simulink model "MIL4L3_SW6_V1_20220211"  (R2018b)
settings: Solver=FixedStepAuto  StartTime=0.0  StopTime=inf  FixedStep=0.001  RelTol=1e-3
PreLoadFcn:
  | A0_MILtest;
undefined symbols (not defined in the file or in its folder): Clb_ICADirect_LaneDisp_StateFive, Clb_ICADirect_LaneDisp_StateFour, Clb_ICADirect_LaneDisp_StateOne, Clb_ICADirect_LaneDisp_StateThree, Clb_ICADirect_LaneDisp_StateTwo, Clb_ICADirect_LaneDisp_StateZero, Clb_ICADirect_LaneDispSW, Clb_ICADirect_TrnLghtsCom_Switch, Clb_ICADirect_TrnLghtsCom_Value, Clb_ICADirect_TrnLghtsCrtl_Inhb, IMAP_Clb_ACU_Driver_Belt, IMAP_Clb_ACU_Driver_Belt_Over, IMAP_Clb_ACU_Passenger_Belt, IMAP_Clb_ACU_Passenger_Belt_Over, IMAP_Clb_ACU_RearLeft_Belt, IMAP_Clb_ACU_RearLeft_Belt_Over, IMAP_Clb_ACU_RearMiddle_Belt, IMAP_Clb_ACU_RearMiddle_Belt_Over, IMAP_Clb_ACU_RearRight_Belt, IMAP_Clb_ACU_RearRight_Belt_Over, IMAP_Clb_AEB_Switch, IMAP_Clb_AEB_Switch_Over, IMAP_Clb_ALC_TLC_Mode, IMAP_Clb_ALC_TLC_Mode_Over, IMAP_Clb_BCM_Battery_Voltage, IMAP_Clb_BCM_Battery_Voltage_Over, IMAP_Clb_BCM_BrakeLamp_State, IMAP_Clb_BCM_BrakeLamp_State_Over, IMAP_Clb_BCM_CHMSL_Status, IMAP_Clb_BCM_CHMSL_Status_Over, IMAP_Clb_BCM_Door_Lock_State, IMAP_Clb_BCM_Door_Lock_State_Over, IMAP_Clb_BCM_FrontWiper_State, IMAP_Clb_BCM_FrontWiper_State_Over, IMAP_Clb_BCM_FrontWiper_Switch, IMAP_Clb_BCM_FrontWiper_Switch_Over, IMAP_Clb_BCM_HazardLamp, IMAP_Clb_BCM_HazardLamp_Over, IMAP_Clb_BCM_HazardLamp_Switch, IMAP_Clb_BCM_HazardLamp_Switch_Over, IMAP_Clb_BCM_HighBeam_State, IMAP_Clb_BCM_HighBeam_State_Over, IMAP_Clb_BCM_Ignition_State, IMAP_Clb_BCM_Ignition_State_Over, IMAP_Clb_BCM_IHBC_Enabled, IMAP_Clb_BCM_IHBC_Enabled_Over, IMAP_Clb_BCM_Left_Light, IMAP_Clb_BCM_Left_Light_Over, IMAP_Clb_BCM_LeftTurn_Switch, IMAP_Clb_BCM_LeftTurn_Switch_Over, IMAP_Clb_BCM_LF_Door_State, IMAP_Clb_BCM_LF_Door_State_Over, IMAP_Clb_BCM_LowBeam_State, IMAP_Clb_BCM_LowBeam_State_Over, IMAP_Clb_BCM_LR_Door_State, IMAP_Clb_BCM_LR_Door_State_Over, IMAP_Clb_BCM_RF_Door_State, IMAP_Clb_BCM_RF_Door_State_Over, IMAP_Clb_BCM_Right_Light, IMAP_Clb_BCM_Right_Light_Over ... (+547)
libraries: CarMaker4SL x2153, simulink x292, dspstat3 x3, canmsglib x2, simulink_extras x1
(part 28 of 52)

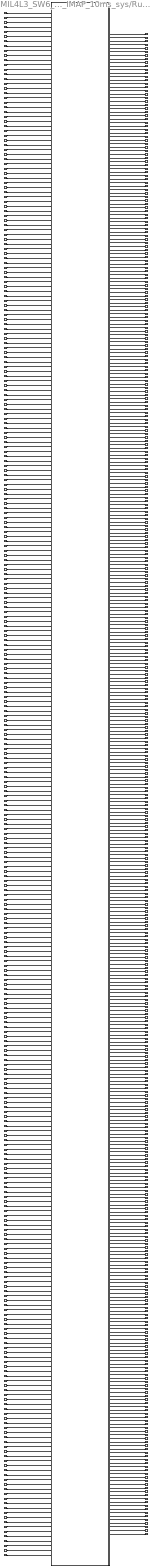
== system MIL4L3_SW6_V1_20220211/CarMaker/VehicleControl/Data Inport/IMAP/Runnable_IMAP_10ms_sys/Runnable_IMAP_10ms_sys ==
  SWINve_y_ABS_in_regulation : Inport  OutDataTypeStr=uint8  PortDimensions=1
  SWINve_g_ACCEL_LONGI_CALIB : Inport  Port=2  OutDataTypeStr=single  PortDimensions=1
  SWINve_y_ASR_ESP_disconnected : Inport  Port=3  OutDataTypeStr=uint8  PortDimensions=1
  SWINve_y_ASR_in_regulation : Inport  Port=4  OutDataTypeStr=uint8  PortDimensions=1
  SWINve_y_BCM_BrakeLampStatus : Inport  Port=5  OutDataTypeStr=uint8  PortDimensions=1
  SWINve_y_BCM_CHMSLStatus : Inport  Port=6  OutDataTypeStr=uint8  PortDimensions=1
  SWINve_y_BCM_State_Front_Wiper : Inport  Port=7  OutDataTypeStr=uint8  PortDimensions=1
  SWINve_y_BCM_Status_Indicator : Inport  Port=8  OutDataTypeStr=uint8  PortDimensions=1
  SWINve_y_Brake_secondary_contact : Inport  Port=9  OutDataTypeStr=uint8  PortDimensions=1
  SWINve_y_Braking_effort : Inport  Port=10  OutDataTypeStr=uint8  PortDimensions=1
  SWINve_y_Dynamic_slope : Inport  Port=11  OutDataTypeStr=int8  PortDimensions=1
  SWINve_y_Dynamic_slope_accuracy : Inport  Port=12  OutDataTypeStr=uint8  PortDimensions=1
  SWINve_y_EMS_ACC_Effecitive_EMS : Inport  Port=13  OutDataTypeStr=uint8  PortDimensions=1
  SWINve_y_EMS_ACCcontrol_Available : Inport  Port=14  OutDataTypeStr=uint8  PortDimensions=1
  SWINve_g_EMS_Acceleration_pedal_position : Inport  Port=15  OutDataTypeStr=single  PortDimensions=1
  SWINve_g_EMS_Actual_torque : Inport  Port=16  OutDataTypeStr=single  PortDimensions=1
  SWINve_g_EMS_Actual_whlTrq : Inport  Port=17  OutDataTypeStr=int16  PortDimensions=1
  SWINve_g_EMS_Driver_request : Inport  Port=18  OutDataTypeStr=single  PortDimensions=1
  SWINve_g_EMS_Driver_wheel_torque : Inport  Port=19  OutDataTypeStr=single  PortDimensions=1
  SWINve_g_EMS_Engine_RPM : Inport  Port=20  OutDataTypeStr=single  PortDimensions=1
  SWINve_y_EMS_Engine_state : Inport  Port=21  OutDataTypeStr=uint8  PortDimensions=1
  SWINve_y_EMS_GearBox_ACC_Ctl_Available : Inport  Port=22  OutDataTypeStr=uint8  PortDimensions=1
  SWINve_g_EMS_WhlTrq_max : Inport  Port=23  OutDataTypeStr=single  PortDimensions=1
  SWINve_g_EMS_WhlTrq_max_offset : Inport  Port=24  OutDataTypeStr=single  PortDimensions=1
  SWINve_g_EMS_WhlTrq_min : Inport  Port=25  OutDataTypeStr=single  PortDimensions=1
  SWINve_g_EMS_WhlTrq_min_offset : Inport  Port=26  OutDataTypeStr=single  PortDimensions=1
  SWINve_y_ESP_in_regulation : Inport  Port=27  OutDataTypeStr=uint8  PortDimensions=1
  SWINve_y_Front_Left_pulse_malfunction : Inport  Port=28  OutDataTypeStr=uint8  PortDimensions=1
  SWINve_y_Front_right_pulse_malfunction : Inport  Port=29  OutDataTypeStr=uint8  PortDimensions=1
  SWINve_y_GW_BCM_SEV_main_state : Inport  Port=30  OutDataTypeStr=uint8  PortDimensions=1
  SWINve_y_GW_EMS_ACC_Ihibited_By_Engine : Inport  Port=31  OutDataTypeStr=uint8  PortDimensions=1
  SWINve_y_GW_EMS_EMS_Status_ACC : Inport  Port=32  OutDataTypeStr=uint8  PortDimensions=1
  SWINve_g_GW_EMS_Pot_WhlTrq_Max : Inport  Port=33  OutDataTypeStr=single  PortDimensions=1
  SWINve_g_GW_EMS_Pot_WhlTrq_Min : Inport  Port=34  OutDataTypeStr=single  PortDimensions=1
  SWINve_y_GW_Mp5_ISA_Switch : Inport  Port=35  OutDataTypeStr=uint8  PortDimensions=1
  SWINve_y_GW_Mp5_TSR_Switch : Inport  Port=36  OutDataTypeStr=uint8  PortDimensions=1
  SWINve_y_GW_SCC_LeftSteeringWheelSwitch : Inport  Port=37  OutDataTypeStr=uint8  PortDimensions=1
  SWINve_y_GW_SCC_RightSteeringWheelSwitch : Inport  Port=38  OutDataTypeStr=uint8  PortDimensions=1
  SWINve_y_BCM_HazardSwitchrSt : Inport  Port=39  OutDataTypeStr=uint8  PortDimensions=1
  SWINve_y_MP5_HazardLampCtrlReq : Inport  Port=40  OutDataTypeStr=uint8  PortDimensions=1
  SWINve_y_T_box_RemoteHazardReq : Inport  Port=41  OutDataTypeStr=uint8  PortDimensions=1
  SWINve_y_High_beam_state : Inport  Port=42  OutDataTypeStr=uint8  PortDimensions=1
  SWINve_y_IC_Fcw_Activation_Config : Inport  Port=43  OutDataTypeStr=uint8  PortDimensions=1
  SWINve_y_IC_FCW_Sensitivity : Inport  Port=44  OutDataTypeStr=uint8  PortDimensions=1
  SWINve_y_IC_passengerBeltSwitchSig : Inport  Port=45  OutDataTypeStr=uint8  PortDimensions=1
  SWINve_y_IC_seat_bealt_driver_state : Inport  Port=46  OutDataTypeStr=uint8  PortDimensions=1
  SWINve_y_Internal_SWS_status : Inport  Port=47  OutDataTypeStr=uint8  PortDimensions=1
  SWINve_g_Lateral_acceleration : Inport  Port=48  OutDataTypeStr=single  PortDimensions=1
  SWINve_y_LC_Mode : Inport  Port=49  OutDataTypeStr=uint8  PortDimensions=1
  SWINve_y_LKA_main_switch : Inport  Port=50  OutDataTypeStr=uint8  PortDimensions=1
  SWINve_y_Message_from_ESC_informing : Inport  Port=51  OutDataTypeStr=uint8  PortDimensions=1
  SWINve_y_MP5_AEB_Activation_Config : Inport  Port=52  OutDataTypeStr=uint8  PortDimensions=1
  SWINve_y_MSR_in_regulation : Inport  Port=53  OutDataTypeStr=uint8  PortDimensions=1
  SWINve_g_No_filtered_front_left_speed : Inport  Port=54  OutDataTypeStr=single  PortDimensions=1
  SWINve_g_No_filtered_front_right_speed : Inport  Port=55  OutDataTypeStr=single  PortDimensions=1
  SWINve_g_No_filtered_rear_left_speed : Inport  Port=56  OutDataTypeStr=single  PortDimensions=1
  SWINve_g_No_filtered_rear_rignt_speed : Inport  Port=57  OutDataTypeStr=single  PortDimensions=1
  SWINve_g_number_of_kilometer : Inport  Port=58  OutDataTypeStr=uint32  PortDimensions=1
  SWINve_y_Park_brake_function_status : Inport  Port=59  OutDataTypeStr=uint8  PortDimensions=1
  SWINve_g_Pulse_counter_front_left_wheel : Inport  Port=60  OutDataTypeStr=uint16  PortDimensions=1
  SWINve_g_Pulse_counter_front_right_wheel : Inport  Port=61  OutDataTypeStr=uint16  PortDimensions=1
  SWINve_g_Pulse_counter_rearleft_wheel : Inport  Port=62  OutDataTypeStr=uint16  PortDimensions=1
  SWINve_g_Pulse_counter_rearright_wheel : Inport  Port=63  OutDataTypeStr=uint16  PortDimensions=1
  SWINve_y_Rear_Left_pulse_malfunction : Inport  Port=64  OutDataTypeStr=uint8  PortDimensions=1
  SWINve_y_Rear_Right_pulse_malfunction : Inport  Port=65  OutDataTypeStr=uint8  PortDimensions=1
  SWINve_y_Request_to_light_fault_lamp : Inport  Port=66  OutDataTypeStr=uint8  PortDimensions=1
  SWINve_y_State_indicating_steer_or_not : Inport  Port=67  OutDataTypeStr=uint8  PortDimensions=1
  SWINve_y_State_of_EPS_for_LKA_function : Inport  Port=68  OutDataTypeStr=uint8  PortDimensions=1
  SWINve_g_Static_slope : Inport  Port=69  OutDataTypeStr=int8  PortDimensions=1
  SWINve_g_Steering_wheel_angle : Inport  Port=70  OutDataTypeStr=single  PortDimensions=1
  SWINve_g_Steering_wheel_rotation_speed : Inport  Port=71  OutDataTypeStr=single  PortDimensions=1
  SWINve_g_Steering_wheel_torque : Inport  Port=72  OutDataTypeStr=single  PortDimensions=1
  SWINve_y_SWS_calibration : Inport  Port=73  OutDataTypeStr=uint8  PortDimensions=1
  SWINve_y_SWS_trim : Inport  Port=74  OutDataTypeStr=uint8  PortDimensions=1
  SWINve_y_TCU_AGB_Target_position : Inport  Port=75  OutDataTypeStr=uint8  PortDimensions=1
  SWINve_y_TCU_ATFailure : Inport  Port=76  OutDataTypeStr=uint8  PortDimensions=1
  SWINve_y_TCU_DCTClutchStatus : Inport  Port=77  OutDataTypeStr=uint8  PortDimensions=1
  SWINve_y_TCU_Gear_lever_position : Inport  Port=78  OutDataTypeStr=uint8  PortDimensions=1
  SWINve_y_TCU_GearEngagement : Inport  Port=79  OutDataTypeStr=uint8  PortDimensions=1
  SWINve_y_TCU_PROGRAMME_ACC : Inport  Port=80  OutDataTypeStr=uint8  PortDimensions=1
  SWINve_g_TMC_pressure : Inport  Port=81  OutDataTypeStr=single  PortDimensions=1
  SWINve_y_Torque_limitation_if_DAE_limit : Inport  Port=82  OutDataTypeStr=uint8  PortDimensions=1
  SWINve_y_Vehicle_detected_as_stationary : Inport  Port=83  OutDataTypeStr=uint8  PortDimensions=1
  SWINve_y_Vehicle_driving_direction : Inport  Port=84  OutDataTypeStr=uint8  PortDimensions=1
  SWINve_y_Vehicle_Hold_Status : Inport  Port=85  OutDataTypeStr=uint8  PortDimensions=1
  SWINve_g_Vehicle_speed_of_wheelsensor : Inport  Port=86  OutDataTypeStr=single  PortDimensions=1
  SWINve_y_Vehiclespd_unavailability_flag : Inport  Port=87  OutDataTypeStr=uint8  PortDimensions=1
  SWINve_g_Yaw_speed : Inport  Port=88  OutDataTypeStr=single  PortDimensions=1
  SWINve_g_YawRate_Raw : Inport  Port=89  OutDataTypeStr=single  PortDimensions=1
  System_Clock : Inport  Port=90  OutDataTypeStr=uint16  PortDimensions=1
  SDFAve_d_sensor_status : Inport  Port=91  OutDataTypeStr=uint16  PortDimensions=1
  SDFAve_d_sen_sta_LF_radar : Inport  Port=92  OutDataTypeStr=uint16  PortDimensions=1
  SDFAve_d_sen_sta_RF_radar : Inport  Port=93  OutDataTypeStr=uint16  PortDimensions=1
  SDFAve_d_sen_sta_LB_radar : Inport  Port=94  OutDataTypeStr=uint16  PortDimensions=1
  SDFAve_d_sen_sta_RB_radar : Inport  Port=95  OutDataTypeStr=uint16  PortDimensions=1
  SDFAve_d_fusion_status : Inport  Port=96  OutDataTypeStr=uint16  PortDimensions=1
  SDFAve_d_fusion_time_stamp : Inport  Port=97  OutDataTypeStr=uint16  PortDimensions=1
  SDFAve_d_obj_Num : Inport  Port=98  OutDataTypeStr=uint16  PortDimensions=1
  SDFAva_y_obj_id : Inport  Port=99  OutDataTypeStr=uint8  PortDimensions=40
  SDFAva_g_obj_pos_x : Inport  Port=100  OutDataTypeStr=single  PortDimensions=40
  SDFAva_g_obj_pos_y : Inport  Port=101  OutDataTypeStr=single  PortDimensions=40
  SDFAva_g_obj_vel_x : Inport  Port=102  OutDataTypeStr=single  PortDimensions=40
  SDFAva_g_obj_vel_y : Inport  Port=103  OutDataTypeStr=single  PortDimensions=40
  SDFAva_g_obj_acc_x : Inport  Port=104  OutDataTypeStr=single  PortDimensions=40
  SDFAva_g_obj_acc_y : Inport  Port=105  OutDataTypeStr=single  PortDimensions=40
  SDFAva_g_obj_pos_var_x : Inport  Port=106  OutDataTypeStr=single  PortDimensions=40
  SDFAva_g_obj_pos_var_y : Inport  Port=107  OutDataTypeStr=single  PortDimensions=40
  SDFAva_g_obj_pos_var_xy : Inport  Port=108  OutDataTypeStr=single  PortDimensions=40
  SDFAva_g_obj_width : Inport  Port=109  OutDataTypeStr=single  PortDimensions=40
  SDFAva_g_obj_length : Inport  Port=110  OutDataTypeStr=single  PortDimensions=40
  SDFAva_y_obj_class : Inport  Port=111  OutDataTypeStr=uint8  PortDimensions=40
  SDFAva_y_obj_lane : Inport  Port=112  OutDataTypeStr=uint8  PortDimensions=40
  SDFAva_d_obj_status : Inport  Port=113  OutDataTypeStr=uint16  PortDimensions=40
  SDFAva_d_obj_age : Inport  Port=114  OutDataTypeStr=uint16  PortDimensions=40
  SDFAva_y_obj_TurnLight : Inport  Port=115  OutDataTypeStr=uint8  PortDimensions=40
  SDFAva_y_obj_BrakeLight : Inport  Port=116  OutDataTypeStr=uint8  PortDimensions=40
  SDFAva_y_obj_MotionStatus : Inport  Port=117  OutDataTypeStr=uint8  PortDimensions=40
  SDFAve_y_ROAD_TYPE : Inport  Port=118  OutDataTypeStr=uint8  PortDimensions=1
  SDFAve_g_L0_C0_COEF : Inport  Port=119  OutDataTypeStr=single  PortDimensions=1
  SDFAve_g_L0_C1_COEF : Inport  Port=120  OutDataTypeStr=single  PortDimensions=1
  SDFAve_g_L0_C2_COEF : Inport  Port=121  OutDataTypeStr=single  PortDimensions=1
  SDFAve_g_L0_C3_COEF : Inport  Port=122  OutDataTypeStr=single  PortDimensions=1
  SDFAve_g_L0_VIEW_RANGE : Inport  Port=123  OutDataTypeStr=single  PortDimensions=1
  SDFAve_y_L0_DETECT_QUALITY : Inport  Port=124  OutDataTypeStr=uint8  PortDimensions=1
  SDFAve_d_L0_LINE_TYPE : Inport  Port=125  OutDataTypeStr=uint16  PortDimensions=1
  SDFAve_g_L0_MARK_WIDTH : Inport  Port=126  OutDataTypeStr=single  PortDimensions=1
  SDFAve_g_R0_C0_COEF : Inport  Port=127  OutDataTypeStr=single  PortDimensions=1
  SDFAve_g_R0_C1_COEF : Inport  Port=128  OutDataTypeStr=single  PortDimensions=1
  SDFAve_g_R0_C2_COEF : Inport  Port=129  OutDataTypeStr=single  PortDimensions=1
  SDFAve_g_R0_C3_COEF : Inport  Port=130  OutDataTypeStr=single  PortDimensions=1
  SDFAve_g_R0_VIEW_RANGE : Inport  Port=131  OutDataTypeStr=single  PortDimensions=1
  SDFAve_y_R0_DETECT_QUALITY : Inport  Port=132  OutDataTypeStr=uint8  PortDimensions=1
  SDFAve_d_R0_LINE_TYPE : Inport  Port=133  OutDataTypeStr=uint16  PortDimensions=1
  SDFAve_g_R0_MARK_WIDTH : Inport  Port=134  OutDataTypeStr=single  PortDimensions=1
  SDFAve_g_L1_C0_COEF : Inport  Port=135  OutDataTypeStr=single  PortDimensions=1
  SDFAve_g_L1_C1_COEF : Inport  Port=136  OutDataTypeStr=single  PortDimensions=1
  SDFAve_g_L1_C2_COEF : Inport  Port=137  OutDataTypeStr=single  PortDimensions=1
  SDFAve_g_L1_C3_COEF : Inport  Port=138  OutDataTypeStr=single  PortDimensions=1
  SDFAve_g_L1_VIEW_RANGE : Inport  Port=139  OutDataTypeStr=single  PortDimensions=1
  SDFAve_y_L1_DETECT_QUALITY : Inport  Port=140  OutDataTypeStr=uint8  PortDimensions=1
  SDFAve_d_L1_LINE_TYPE : Inport  Port=141  OutDataTypeStr=uint16  PortDimensions=1
  SDFAve_g_L1_MARK_WIDTH : Inport  Port=142  OutDataTypeStr=single  PortDimensions=1
  SDFAve_g_R1_C0_COEF : Inport  Port=143  OutDataTypeStr=single  PortDimensions=1
  SDFAve_g_R1_C1_COEF : Inport  Port=144  OutDataTypeStr=single  PortDimensions=1
  SDFAve_g_R1_C2_COEF : Inport  Port=145  OutDataTypeStr=single  PortDimensions=1
  SDFAve_g_R1_C3_COEF : Inport  Port=146  OutDataTypeStr=single  PortDimensions=1
  SDFAve_g_R1_VIEW_RANGE : Inport  Port=147  OutDataTypeStr=single  PortDimensions=1
  SDFAve_y_R1_DETECT_QUALITY : Inport  Port=148  OutDataTypeStr=uint8  PortDimensions=1
  SDFAve_d_R1_LINE_TYPE : Inport  Port=149  OutDataTypeStr=uint16  PortDimensions=1
  SDFAve_g_R1_MARK_WIDTH : Inport  Port=150  OutDataTypeStr=single  PortDimensions=1
  SDFAve_g_L0_C0_BACK_COEF : Inport  Port=151  OutDataTypeStr=single  PortDimensions=1
  SDFAve_g_L0_C1_BACK_COEF : Inport  Port=152  OutDataTypeStr=single  PortDimensions=1
  SDFAve_g_L0_C2_BACK_COEF : Inport  Port=153  OutDataTypeStr=single  PortDimensions=1
  SDFAve_g_L0_C3_BACK_COEF : Inport  Port=154  OutDataTypeStr=single  PortDimensions=1
  SDFAve_g_L0_BACK_RANGE : Inport  Port=155  OutDataTypeStr=single  PortDimensions=1
  SDFAve_g_R0_C0_BACK_COEF : Inport  Port=156  OutDataTypeStr=single  PortDimensions=1
  SDFAve_g_R0_C1_BACK_COEF : Inport  Port=157  OutDataTypeStr=single  PortDimensions=1
  SDFAve_g_R0_C2_BACK_COEF : Inport  Port=158  OutDataTypeStr=single  PortDimensions=1
  SDFAve_g_R0_C3_BACK_COEF : Inport  Port=159  OutDataTypeStr=single  PortDimensions=1
  SDFAve_g_R0_BACK_RANGE : Inport  Port=160  OutDataTypeStr=single  PortDimensions=1
  SDFAve_g_L1_C0_BACK_COEF : Inport  Port=161  OutDataTypeStr=single  PortDimensions=1
  SDFAve_g_L1_C1_BACK_COEF : Inport  Port=162  OutDataTypeStr=single  PortDimensions=1
  SDFAve_g_L1_C2_BACK_COEF : Inport  Port=163  OutDataTypeStr=single  PortDimensions=1
  SDFAve_g_L1_C3_BACK_COEF : Inport  Port=164  OutDataTypeStr=single  PortDimensions=1
  SDFAve_g_L1_BACK_RANGE : Inport  Port=165  OutDataTypeStr=single  PortDimensions=1
  SDFAve_g_R1_C0_BACK_COEF : Inport  Port=166  OutDataTypeStr=single  PortDimensions=1
  SDFAve_g_R1_C1_BACK_COEF : Inport  Port=167  OutDataTypeStr=single  PortDimensions=1
  SDFAve_g_R1_C2_BACK_COEF : Inport  Port=168  OutDataTypeStr=single  PortDimensions=1
  SDFAve_g_R1_C3_BACK_COEF : Inport  Port=169  OutDataTypeStr=single  PortDimensions=1
  SDFAve_g_R1_BACK_RANGE : Inport  Port=170  OutDataTypeStr=single  PortDimensions=1
  SDFAve_g_Lrg_C0_BACK_COEF : Inport  Port=171  OutDataTypeStr=single
  SDFAve_g_Lrg_C1_BACK_COEF : Inport  Port=172  OutDataTypeStr=single
  SDFAve_g_Lrg_C2_BACK_COEF : Inport  Port=173  OutDataTypeStr=single
  SDFAve_g_Lrg_C3_BACK_COEF : Inport  Port=174  OutDataTypeStr=single
  SDFAve_g_Lrg_VIEW_RANGE_start : Inport  Port=175  OutDataTypeStr=single
  SDFAve_g_Lrg_VIEW_RANGE_end : Inport  Port=176  OutDataTypeStr=single
  SDFAve_y_Lrg_DETECT_QUALITY : Inport  Port=177  OutDataTypeStr=uint8
  SDFAve_y_Lrg_LINE_TYPE : Inport  Port=178  OutDataTypeStr=uint8
  SDFAve_g_Rrg_C0_BACK_COEF : Inport  Port=179  OutDataTypeStr=single
  SDFAve_g_Rrg_C1_BACK_COEF : Inport  Port=180  OutDataTypeStr=single
  SDFAve_g_Rrg_C2_BACK_COEF : Inport  Port=181  OutDataTypeStr=single
  SDFAve_g_Rrg_C3_BACK_COEF : Inport  Port=182  OutDataTypeStr=single
  SDFAve_g_Rrg_VIEW_RANGE_start : Inport  Port=183  OutDataTypeStr=single
  SDFAve_g_Rrg_VIEW_RANGE_end : Inport  Port=184  OutDataTypeStr=single
  SDFAve_y_Rrg_DETECT_QUALITY : Inport  Port=185  OutDataTypeStr=uint8
  SDFAve_y_Rrg_LINE_TYPE : Inport  Port=186  OutDataTypeStr=uint8
  SDFAve_y_ISAValue : Inport  Port=187  OutDataTypeStr=uint8  PortDimensions=1
  SDFAve_y_ISAPopupMessage : Inport  Port=188  OutDataTypeStr=uint8
  SDFAve_y_ISASignType : Inport  Port=189  OutDataTypeStr=uint8
  SDFAve_y_ISAStatus : Inport  Port=190  OutDataTypeStr=uint8
  SDFAve_y_TSR_Sign_Type : Inport  Port=191  OutDataTypeStr=uint8  PortDimensions=1
  SDFAve_g_CameraSignalFault : Inport  Port=192  OutDataTypeStr=single  PortDimensions=1
  SDFAve_y_Radar_State : Inport  Port=193  OutDataTypeStr=uint8  PortDimensions=1
  SDFAve_y_OperatingStatus : Inport  Port=194  OutDataTypeStr=uint8  PortDimensions=1
  SDFAve_y_Radar_FaultBitSetting_Signal : Inport  Port=195
  SWINve_y_ESC_FLWDirection : Inport  Port=196  OutDataTypeStr=uint8  PortDimensions=1
  SWINve_y_ESC_FRWDirection : Inport  Port=197  OutDataTypeStr=uint8  PortDimensions=1
  SWINve_y_ESC_TCSErrorStatus : Inport  Port=198  OutDataTypeStr=uint8  PortDimensions=1
  SWINve_y_ESC-RLWDirection : Inport  Port=199  OutDataTypeStr=uint8  PortDimensions=1
  SWINve_y_ESC_RRWDirection : Inport  Port=200  OutDataTypeStr=uint8  PortDimensions=1
  SWINve_y_ESC_EPBErrorStatus : Inport  Port=201  OutDataTypeStr=uint8  PortDimensions=1
  SWINve_y_EPS_SteeringAngle_Flag : Inport  Port=202  OutDataTypeStr=uint8  PortDimensions=1
  SWINve_g_EPS_SteeringAngle : Inport  Port=203  OutDataTypeStr=single  PortDimensions=1
  SWINve_y_EPS_DriverOverride : Inport  Port=204  OutDataTypeStr=uint8  PortDimensions=1
  SWINve_y_EPS_DriverInitializedESA : Inport  Port=205  OutDataTypeStr=uint8
  SWINve_y_EPS_ESAState : Inport  Port=206  OutDataTypeStr=uint8
  SWINve_y_ACU_RearLeftBeltSwitchSig : Inport  Port=207  OutDataTypeStr=uint8
  SWINve_y_ACU_RearMiddleBeltSwitchSig : Inport  Port=208  OutDataTypeStr=uint8
  SWINve_y_ACU_RearRightBeltSwitchSig : Inport  Port=209  OutDataTypeStr=uint8
  SWINve_y_EMS_PowertrainControlSt : Inport  Port=210  OutDataTypeStr=uint8
  SWINve_y_TCU_TCUAvailable : Inport  Port=211  OutDataTypeStr=uint8
  SWINve_y_BCM_LeftTurnSwitchSt : Inport  Port=212  OutDataTypeStr=uint8
  SWINve_y_BCM_RightTurnSwitchSt : Inport  Port=213  OutDataTypeStr=uint8
  SWINve_y_BCM_FrontWiperSwitchSt : Inport  Port=214  OutDataTypeStr=uint8
  SWINve_y_BCM_IHBC_Function_Enabled : Inport  Port=215  OutDataTypeStr=uint8
  SWINve_y_MP5_WorkSt : Inport  Port=216  OutDataTypeStr=uint8
  SWINve_y_MP5_APAModeSelect : Inport  Port=217  OutDataTypeStr=uint8
  SWINve_y_MP5_LanguageSet : Inport  Port=218  OutDataTypeStr=uint8
  SWINve_y_MP5_UPASwitch : Inport  Port=219  OutDataTypeStr=uint8
  SWINve_y_MP5_FLKActivation : Inport  Port=220  OutDataTypeStr=uint8
  SWINve_y_MP5_AutoPilotSwitch : Inport  Port=221  OutDataTypeStr=uint8
  SWINve_y_MP5_DMS_MessageType : Inport  Port=222  OutDataTypeStr=uint8
  SWINve_y_MP5_DMS_SystemEnable : Inport  Port=223  OutDataTypeStr=uint8
  SWINve_y_MP5_DMS_DeleteUserNum : Inport  Port=224  OutDataTypeStr=uint8
  SWINve_y_MP5_DMS_Sensity : Inport  Port=225  OutDataTypeStr=uint8
  SWINve_y_MP5_DMS_EyeFatigueMonitor : Inport  Port=226  OutDataTypeStr=uint8
  SWINve_y_MP5_DMS_LongtimeDriveMonitor : Inport  Port=227  OutDataTypeStr=uint8
  SWINve_y_MP5_DMS_SideViewMonitor : Inport  Port=228  OutDataTypeStr=uint8
  SWINve_y_MP5_DMS_UsingPhoneMonitor : Inport  Port=229  OutDataTypeStr=uint8
  SWINve_y_MP5_DMS_SmokingMonitor : Inport  Port=230  OutDataTypeStr=uint8
  SWINve_y_MP5_DMS_DrinkWaterMonitor : Inport  Port=231  OutDataTypeStr=uint8
  SWINve_y_MP5_DMS_UserAccount : Inport  Port=232  OutDataTypeStr=uint8
  SWINve_y_Mp5_ISAMode : Inport  Port=233  OutDataTypeStr=uint8  PortDimensions=1
  SWINve_y_Mp5_LDWWarningMode : Inport  Port=234  OutDataTypeStr=uint8  PortDimensions=1
  SWINve_y_MP5_ADASSpeedLimit : Inport  Port=235  OutDataTypeStr=uint8  PortDimensions=1
  SWINve_y_MP5_TLCModeSelection : Inport  Port=236  OutDataTypeStr=uint8  PortDimensions=1
  SWINve_y_MP5_ESASwitch : Inport  Port=237  OutDataTypeStr=uint8  PortDimensions=1
  SWINve_y_Mp5_ELKSwitch : Inport  Port=238  OutDataTypeStr=uint8  PortDimensions=1
  SWINve_y_PEPS_RKECommand : Inport  Port=239  OutDataTypeStr=uint8  PortDimensions=1
  SWINve_y_MP5_BSD_LCW_Activation : Inport  Port=240  OutDataTypeStr=uint8  PortDimensions=1
  SWINve_y_MP5_FCTAActivation : Inport  Port=241  OutDataTypeStr=uint8  PortDimensions=1
  SWINve_y_MP5_RCTAActivation : Inport  Port=242  OutDataTypeStr=uint8  PortDimensions=1
  SWINve_y_MP5_DOWActivation : Inport  Port=243  OutDataTypeStr=uint8
  SWINve_y_MP5_JA_Modes : Inport  Port=244  OutDataTypeStr=uint8
  SWINve_y_MP5_JA_Alert_Switch : Inport  Port=245  OutDataTypeStr=uint8
  SWINve_y_ESC_BLRequest : Inport  Port=246  OutDataTypeStr=uint8  PortDimensions=1
  SWINve_y_PEPS_DoorLockReq : Inport  Port=247  OutDataTypeStr=uint8  PortDimensions=1
  SWINve_y_BCM_DoorLockSt : Inport  Port=248  OutDataTypeStr=uint8  PortDimensions=1
  SWINve_y_BCM_LowBeamStatus : Inport  Port=249  OutDataTypeStr=uint8  PortDimensions=1
  SWINve_g_BCM_BattVolt : Inport  Port=250  OutDataTypeStr=single  PortDimensions=1
  SWINve_d_TBOX_LocalTimeYear : Inport  Port=251  OutDataTypeStr=uint16  PortDimensions=1
  SWINve_y_TBOX_LocalTimeMonth : Inport  Port=252  OutDataTypeStr=uint8  PortDimensions=1
  SWINve_y_TBOX_LocalTimeDate : Inport  Port=253  OutDataTypeStr=uint8  PortDimensions=1
  SWINve_y_TBOX_LocalTimeHour : Inport  Port=254  OutDataTypeStr=uint8  PortDimensions=1
  SWINve_y_TBOX_LocalTimeMinute : Inport  Port=255  OutDataTypeStr=uint8
  SWINve_y_TBOX_LocalTimeSecond : Inport  Port=256  OutDataTypeStr=uint8
  SWINve_y_TBOX_LocalTimeValid : Inport  Port=257  OutDataTypeStr=uint8
  SWINve_g_AC_AmbTemp : Inport  Port=258  OutDataTypeStr=single
  SWINve_y_EPS_SteeringTorqueSensorSt : Inport  Port=259  OutDataTypeStr=uint8  PortDimensions=1
  SWINve_g_EPS_LKACurrentOverlay : Inport  Port=260  OutDataTypeStr=single  PortDimensions=1
  SWINve_y_EPS_WarningLampSt : Inport  Port=261  OutDataTypeStr=uint8  PortDimensions=1
  SWINve_g_EPS_ElectPowerConsumption : Inport  Port=262  OutDataTypeStr=single  PortDimensions=1
  SWINve_g_EMS_EngActualIndTorque : Inport  Port=263  OutDataTypeStr=single  PortDimensions=1
  SWINve_y_EMS_AccPedalFaultBit : Inport  Port=264  OutDataTypeStr=uint8  PortDimensions=1
  SWINve_y_TCU_PRNDLStatus : Inport  Port=265  OutDataTypeStr=uint8  PortDimensions=1
  SWINve_y_TCU_ShiftLeverPosValidFlag : Inport  Port=266  OutDataTypeStr=uint8  PortDimensions=1
  SWINve_y_ESC_LateralAccelarationValidity : Inport  Port=267  OutDataTypeStr=uint8  PortDimensions=1
  SWINve_y_ESC_YawrateValidity : Inport  Port=268  OutDataTypeStr=uint8
  SWINve_y_ESC_LongitudinalAccelerationValidity : Inport  Port=269  OutDataTypeStr=uint8
  SWINve_y_ESC_ABSValidity : Inport  Port=270  OutDataTypeStr=uint8
  SWINve_y_ESC_ABSAlarmSig : Inport  Port=271  OutDataTypeStr=uint8
  SWINve_y_ESC_FLWHeelSpdFaultSignal : Inport  Port=272  OutDataTypeStr=uint8
  SWINve_y_ESC_FRWHeelSpdFaultSignal : Inport  Port=273  OutDataTypeStr=uint8
  SWINve_y_ESC_RLWHeelSpdFaultSignal : Inport  Port=274  OutDataTypeStr=uint8
  SWINve_y_ESC_RRWHeelSpdFaultSignal : Inport  Port=275  OutDataTypeStr=uint8
  SWINve_y_ESC_AEBAvailable : Inport  Port=276  OutDataTypeStr=uint8
  SWINve_y_ESC_AEBActive : Inport  Port=277  OutDataTypeStr=uint8
  SWINve_y_ESC_ACCAvailable : Inport  Port=278  OutDataTypeStr=uint8
  SWINve_y_ESC_ACCActive : Inport  Port=279  OutDataTypeStr=uint8
  SWINve_y_ESC_EPBDisplayMessageReq : Inport  Port=280  OutDataTypeStr=uint8
  SWINve_y_ESC_EPBWarningIndicationReq : Inport  Port=281  OutDataTypeStr=uint8
  SWINve_y_ESC_EPBSwitchStatics : Inport  Port=282  OutDataTypeStr=uint8
  SWINve_y_ESC_EPBSwitchStaticsValidity : Inport  Port=283  OutDataTypeStr=uint8
  SWINve_y_ESC_EBDAlarmSig : Inport  Port=284  OutDataTypeStr=uint8
  SWINve_y_ESC_AVHStatus : Inport  Port=285  OutDataTypeStr=uint8
  SWINve_y_BCM_LeftlightSt : Inport  Port=286  OutDataTypeStr=uint8  PortDimensions=1
  SWINve_y_BCM_RightlightSt : Inport  Port=287  OutDataTypeStr=uint8  PortDimensions=1
  SWINve_y_BCM_TrunkSt : Inport  Port=288  OutDataTypeStr=uint8  PortDimensions=1
  SWINve_y_BCM_LFDoorSwitchSt : Inport  Port=289  OutDataTypeStr=uint8  PortDimensions=1
  SWINve_y_BCM_RFDoorSwitchSt : Inport  Port=290  OutDataTypeStr=uint8  PortDimensions=1
  SWINve_y_BCM_RRDoorSwitchSt : Inport  Port=291  OutDataTypeStr=uint8  PortDimensions=1
  SWINve_y_BCM_LRDoorSwitchSt : Inport  Port=292  OutDataTypeStr=uint8  PortDimensions=1
  SWINve_g_ESC_BrakeWheelCylinderPressure : Inport  Port=293  OutDataTypeStr=single  PortDimensions=1
  FAPAve_Cnt_AdvancedParkingAssist : Inport  Port=294  OutDataTypeStr=uint8
  SDFAve_d_ORI_CIPV_ID : Inport  Port=295  OutDataTypeStr=uint16
  SDFAve_d_ORI_Obj_Num : Inport  Port=296  OutDataTypeStr=uint16
  SDFAva_d_ORI_Obj_Class : Inport  Port=297  OutDataTypeStr=uint16  PortDimensions=20
  SDFAva_d_ORI_Obj_ID : Inport  Port=298  OutDataTypeStr=uint16  PortDimensions=20
  SDFAva_g_ORI_Obj_AbsAx : Inport  Port=299  OutDataTypeStr=single  PortDimensions=20
  SDFAva_g_ORI_Obj_AbsAy : Inport  Port=300  OutDataTypeStr=single  PortDimensions=20
  SDFAva_g_ORI_Obj_RelVel : Inport  Port=301  OutDataTypeStr=single  PortDimensions=20
  SDFAva_g_ORI_Obj_RelVely : Inport  Port=302  OutDataTypeStr=single  PortDimensions=20
  SDFAva_g_ORI_Obj_LongDis : Inport  Port=303  OutDataTypeStr=single  PortDimensions=20
  SDFAva_g_ORI_Obj_LateralDis : Inport  Port=304  OutDataTypeStr=single  PortDimensions=20
  SDFAve_g_ORI_L0_C3 : Inport  Port=305  OutDataTypeStr=single
  SDFAve_g_ORI_L0_C2 : Inport  Port=306  OutDataTypeStr=single
  SDFAve_g_ORI_L0_C1 : Inport  Port=307  OutDataTypeStr=single
  SDFAve_g_ORI_L0_C0 : Inport  Port=308  OutDataTypeStr=single
  SDFAve_d_ORI_L0_Type : Inport  Port=309  OutDataTypeStr=uint16
  SDFAve_g_ORI_L0_VR : Inport  Port=310  OutDataTypeStr=single
  SDFAve_g_ORI_L1_C3 : Inport  Port=311  OutDataTypeStr=single
  SDFAve_g_ORI_L1_C2 : Inport  Port=312  OutDataTypeStr=single
  SDFAve_g_ORI_L1_C1 : Inport  Port=313  OutDataTypeStr=single
  SDFAve_g_ORI_L1_C0 : Inport  Port=314  OutDataTypeStr=single
  SDFAve_d_ORI_L1_Type : Inport  Port=315  OutDataTypeStr=uint16
  SDFAve_g_ORI_L1_VR : Inport  Port=316  OutDataTypeStr=single
  SDFAve_g_ORI_R0_C3 : Inport  Port=317  OutDataTypeStr=single
  SDFAve_g_ORI_R0_C2 : Inport  Port=318  OutDataTypeStr=single
  SDFAve_g_ORI_R0_C1 : Inport  Port=319  OutDataTypeStr=single
  SDFAve_g_ORI_R0_C0 : Inport  Port=320  OutDataTypeStr=single
  SDFAve_d_ORI_R0_LT : Inport  Port=321  OutDataTypeStr=uint16
  SDFAve_g_ORI_R0_VR : Inport  Port=322  OutDataTypeStr=single
  SDFAve_g_ORI_R1_C3 : Inport  Port=323  OutDataTypeStr=single
  SDFAve_g_ORI_R1_C2 : Inport  Port=324  OutDataTypeStr=single
  SDFAve_g_ORI_R1_C1 : Inport  Port=325  OutDataTypeStr=single
  SDFAve_g_ORI_R1_C0 : Inport  Port=326  OutDataTypeStr=single
  SDFAve_d_ORI_R1_LT : Inport  Port=327  OutDataTypeStr=uint16
  SDFAve_g_ORI_R1_VR : Inport  Port=328  OutDataTypeStr=single
  IMAP_Module : Subsystem  TreatAsAtomicUnit=on
  IMAPve_d_LKA_Main_Switch : Outport  OutDataTypeStr=uint16  PortDimensions=1
  IMAPve_d_LKA_Mode : Outport  Port=2  OutDataTypeStr=uint16  PortDimensions=1
  IMAPve_d_AEB_Switch : Outport  Port=3  OutDataTypeStr=uint16  PortDimensions=1
  IMAPve_d_FCW_Switch : Outport  Port=4  OutDataTypeStr=uint16  PortDimensions=1
  IMAPve_d_FCW_Sensitivity : Outport  Port=5  OutDataTypeStr=uint16  PortDimensions=1
  IMAPve_d_ISA_Switch : Outport  Port=6  OutDataTypeStr=uint16  PortDimensions=1
  IMAPve_d_TSR_Switch : Outport  Port=7  OutDataTypeStr=uint16  PortDimensions=1
  IMAPve_d_ISA_ISLC_Mode : Outport  Port=8  OutDataTypeStr=uint16  PortDimensions=1
  IMAPve_d_LDW_Warn_Mode : Outport  Port=9  OutDataTypeStr=uint16  PortDimensions=1
  IMAPve_d_Speed_Limit : Outport  Port=10  OutDataTypeStr=uint16  PortDimensions=1
  IMAPve_d_ALC_TLC_Mode : Outport  Port=11  OutDataTypeStr=uint16  PortDimensions=1
  IMAPve_d_ESA_Switch : Outport  Port=12  OutDataTypeStr=uint16  PortDimensions=1
  IMAPve_d_ELK_Switch : Outport  Port=13  OutDataTypeStr=uint16  PortDimensions=1
  IMAPve_d_PEPS_RKE_Command : Outport  Port=14  OutDataTypeStr=uint16  PortDimensions=1
  IMAPve_d_BSD_LCW_Switch : Outport  Port=15  OutDataTypeStr=uint16  PortDimensions=1
  IMAPve_d_FCTA_Switch : Outport  Port=16  OutDataTypeStr=uint16  PortDimensions=1
  IMAPve_d_RCTA_Swtich : Outport  Port=17  OutDataTypeStr=uint16  PortDimensions=1
  IMAPve_d_DOW_Switch : Outport  Port=18  OutDataTypeStr=uint16  PortDimensions=1
  IMAPve_d_JA_Brake_Switch : Outport  Port=19  OutDataTypeStr=uint16  PortDimensions=1
  IMAPve_d_JA_Alert_Switch : Outport  Port=20  OutDataTypeStr=uint16  PortDimensions=1
  IMAPve_d_EPS_LKA_State : Outport  Port=21  OutDataTypeStr=uint16  PortDimensions=1
  IMAPve_g_EPS_SW_Trq : Outport  Port=22  OutDataTypeStr=single  PortDimensions=1
  IMAPve_d_EPS_Trq_State : Outport  Port=23  OutDataTypeStr=uint16  PortDimensions=1
  IMAPve_d_SAS_Clb_State : Outport  Port=24  OutDataTypeStr=uint16  PortDimensions=1
  IMAPve_d_SAS_Trim_State : Outport  Port=25  OutDataTypeStr=uint16  PortDimensions=1
  IMAPve_d_EPS_TrqLim_State : Outport  Port=26  OutDataTypeStr=uint16  PortDimensions=1
  IMAPve_g_EPS_LKA_Current : Outport  Port=27  OutDataTypeStr=single  PortDimensions=1
  IMAPve_g_ESC_LatAcc : Outport  Port=28  OutDataTypeStr=single  PortDimensions=1
  IMAPve_d_ESC_LatAcc_Valid : Outport  Port=29  OutDataTypeStr=uint16  PortDimensions=1
  IMAPve_g_ESC_YawRate : Outport  Port=30  OutDataTypeStr=single  PortDimensions=1
  IMAPve_d_ESC_YawRate_Valid : Outport  Port=31  OutDataTypeStr=uint16  PortDimensions=1
  IMAPve_g_ESC_UnYawRate : Outport  Port=32  OutDataTypeStr=single  PortDimensions=1
  IMAPve_g_ESC_VehSpd : Outport  Port=33  OutDataTypeStr=single  PortDimensions=1
  IMAPve_g_ESC_LonAcc : Outport  Port=34  OutDataTypeStr=single  PortDimensions=1
  IMAPve_d_ESC_LonAcc_Valid : Outport  Port=35  OutDataTypeStr=uint16  PortDimensions=1
  IMAPve_g_ESC_Brake_Press : Outport  Port=36  OutDataTypeStr=single  PortDimensions=1
  IMAPve_g_ESC_Static_Slope : Outport  Port=37  OutDataTypeStr=single  PortDimensions=1
  IMAPve_g_ESC_DySlope_Accuracy : Outport  Port=38  OutDataTypeStr=single  PortDimensions=1
  IMAPve_g_ESC_DySlope : Outport  Port=39  OutDataTypeStr=single  PortDimensions=1
  IMAPve_g_SW_Angle : Outport  Port=40  OutDataTypeStr=single  PortDimensions=1
  IMAPve_g_SW_Angle_Speed : Outport  Port=41  OutDataTypeStr=single  PortDimensions=1
  IMAPve_d_BCM_HazardLamp : Outport  Port=42  OutDataTypeStr=uint16  PortDimensions=1
  IMAPve_d_BCM_Left_Light : Outport  Port=43  OutDataTypeStr=uint16  PortDimensions=1
  IMAPve_d_BCM_Right_Light : Outport  Port=44  OutDataTypeStr=uint16  PortDimensions=1
  IMAPve_d_ESC_BrakeLamp_Req : Outport  Port=45  OutDataTypeStr=uint16  PortDimensions=1
  IMAPve_d_BCM_Opening_State : Outport  Port=46  OutDataTypeStr=uint16  PortDimensions=1
  IMAPve_d_BCM_Trunk_State : Outport  Port=47  OutDataTypeStr=uint16  PortDimensions=1
  IMAPve_d_BCM_LF_Door_State : Outport  Port=48  OutDataTypeStr=uint16  PortDimensions=1
  IMAPve_d_BCM_RF_Door_State : Outport  Port=49  OutDataTypeStr=uint16  PortDimensions=1
  IMAPve_d_BCM_RR_Door_State : Outport  Port=50  OutDataTypeStr=uint16  PortDimensions=1
  IMAPve_d_BCM_LR_Door_State : Outport  Port=51  OutDataTypeStr=uint16  PortDimensions=1
  IMAPve_d_SCC_Left_SwitchSig : Outport  Port=52  OutDataTypeStr=uint16  PortDimensions=1
  IMAPve_d_SCC_Right_SwitchSig : Outport  Port=53  OutDataTypeStr=uint16  PortDimensions=1
  IMAPve_d_BCM_HazardLamp_Switch : Outport  Port=54
  IMAPve_d_PEPS_Door_Lock_Req : Outport  Port=55  OutDataTypeStr=uint16  PortDimensions=1
  IMAPve_d_BCM_Door_Lock_State : Outport  Port=56  OutDataTypeStr=uint16  PortDimensions=1
  IMAPve_d_EMS_ACC_Status : Outport  Port=57  OutDataTypeStr=uint16  PortDimensions=1
  IMAPve_g_EMS_Pot_WhlT_Max : Outport  Port=58  OutDataTypeStr=single  PortDimensions=1
  IMAPve_g_EMS_Pot_WhlT_Min : Outport  Port=59  OutDataTypeStr=single  PortDimensions=1
  IMAPve_g_EMS_RealPedal : Outport  Port=60  OutDataTypeStr=single  PortDimensions=1
  IMAPve_g_EMS_MaxTWhl : Outport  Port=61  OutDataTypeStr=single  PortDimensions=1
  IMAPve_g_EMS_MaxTWhl_Offset : Outport  Port=62  OutDataTypeStr=single  PortDimensions=1
  IMAPve_g_EMS_MinTWhl : Outport  Port=63  OutDataTypeStr=single  PortDimensions=1
  IMAPve_g_EMS_MinTWhl_Offset : Outport  Port=64  OutDataTypeStr=single  PortDimensions=1
  IMAPve_g_EMS_Actual_FlwT : Outport  Port=65  OutDataTypeStr=single  PortDimensions=1
  IMAPve_g_EMS_Actual_IndT : Outport  Port=66  OutDataTypeStr=single  PortDimensions=1
  IMAPve_g_EMS_Realize_TWhl : Outport  Port=67  OutDataTypeStr=single  PortDimensions=1
  IMAPve_g_EMS_ACC_VirtualPedal : Outport  Port=68  OutDataTypeStr=single  PortDimensions=1
  IMAPve_d_EMS_AccPedal_Fault : Outport  Port=69  OutDataTypeStr=uint16  PortDimensions=1
  IMAPve_g_EMS_Driver_Torque : Outport  Port=70  OutDataTypeStr=single  PortDimensions=1
  IMAPve_d_ESC_Brake_Effort : Outport  Port=71  OutDataTypeStr=uint16  PortDimensions=1
  IMAPve_g_EMS_Engine_Speed : Outport  Port=72  OutDataTypeStr=single  PortDimensions=1
  IMAPve_d_ESC_Veh_Standstill : Outport  Port=73  OutDataTypeStr=uint16  PortDimensions=1
  IMAPve_d_TCU_Actual_Gear : Outport  Port=74  OutDataTypeStr=uint16  PortDimensions=1
  IMAPve_d_TCU_Target_Gear : Outport  Port=75  OutDataTypeStr=uint16  PortDimensions=1
  IMAPve_d_TCU_PRND_State : Outport  Port=76  OutDataTypeStr=uint16  PortDimensions=1
  IMAPve_d_BCM_Ignition_State : Outport  Port=77  OutDataTypeStr=uint16  PortDimensions=1
  IMAPve_d_ACU_Driver_Belt : Outport  Port=78  OutDataTypeStr=uint16  PortDimensions=1
  IMAPve_d_SWS_Failure_Status : Outport  Port=79  OutDataTypeStr=uint16  PortDimensions=1
  IMAPve_d_ESC_OFF : Outport  Port=80  OutDataTypeStr=uint16  PortDimensions=1
  IMAPve_d_ESC_AlarmSig : Outport  Port=81  OutDataTypeStr=uint16  PortDimensions=1
  IMAPve_d_ESC_ESC_Active : Outport  Port=82  OutDataTypeStr=uint16  PortDimensions=1
  IMAPve_d_ESC_MSR_Active : Outport  Port=83  OutDataTypeStr=uint16  PortDimensions=1
  IMAPve_d_ESC_TCS_Active : Outport  Port=84  OutDataTypeStr=uint16  PortDimensions=1
  IMAPve_d_ESC_VehSpd_Valid : Outport  Port=85  OutDataTypeStr=uint16  PortDimensions=1
  IMAPve_d_ESC_ABS_Active : Outport  Port=86  OutDataTypeStr=uint16  PortDimensions=1
  IMAPve_d_ESC_ABS_Valid : Outport  Port=87  OutDataTypeStr=uint16  PortDimensions=1
  IMAPve_d_ESC_ABS_AlarmSig : Outport  Port=88  OutDataTypeStr=uint16  PortDimensions=1
  IMAPve_d_ESC_FL_WheelPulVal : Outport  Port=89  OutDataTypeStr=uint16  PortDimensions=1
  IMAPve_d_ESC_FR_WheelPulVal : Outport  Port=90  OutDataTypeStr=uint16  PortDimensions=1
  IMAPve_d_ESC_RL_WheelPulVal : Outport  Port=91  OutDataTypeStr=uint16  PortDimensions=1
  IMAPve_d_ESC_RR_WheelPulVal : Outport  Port=92  OutDataTypeStr=uint16  PortDimensions=1
  IMAPve_g_ESC_FL_WhlSpd : Outport  Port=93  OutDataTypeStr=single  PortDimensions=1
  IMAPve_d_ESC_FL_WhlSpd_Fault : Outport  Port=94  OutDataTypeStr=uint16  PortDimensions=1
  IMAPve_g_ESC_FR_WhlSpd : Outport  Port=95  OutDataTypeStr=single  PortDimensions=1
  IMAPve_d_ESC_FR_WhlSpd_Fault : Outport  Port=96  OutDataTypeStr=uint16  PortDimensions=1
  IMAPve_g_ESC_RL_WhlSpd : Outport  Port=97  OutDataTypeStr=single  PortDimensions=1
  IMAPve_d_ESC_RL_WhlSpd_Fault : Outport  Port=98  OutDataTypeStr=uint16  PortDimensions=1
  IMAPve_g_ESC_RR_WhlSpd : Outport  Port=99  OutDataTypeStr=single  PortDimensions=1
  IMAPve_d_ESC_RR_WhlSpd_Fault : Outport  Port=100  OutDataTypeStr=uint16  PortDimensions=1
  IMAPve_d_ESC_FL_Wheel_Pulse : Outport  Port=101  OutDataTypeStr=uint16  PortDimensions=1
  IMAPve_d_ESC_FR_Wheel_Pulse : Outport  Port=102  OutDataTypeStr=uint16  PortDimensions=1
  IMAPve_d_ESC_RL_Wheel_Pulse : Outport  Port=103  OutDataTypeStr=uint16  PortDimensions=1
  IMAPve_d_ESC_RR_Wheel_Pulse : Outport  Port=104  OutDataTypeStr=uint16  PortDimensions=1
  IMAPve_d_TCU_AT_Failure : Outport  Port=105  OutDataTypeStr=uint16  PortDimensions=1
  IMAPve_d_TCU_Shift_Valid : Outport  Port=106  OutDataTypeStr=uint16  PortDimensions=1
  IMAPve_d_TCU_DCT_Clutch_State : Outport  Port=107  OutDataTypeStr=uint16  PortDimensions=1
  IMAPve_d_TCU_Gear_Engage : Outport  Port=108  OutDataTypeStr=uint16  PortDimensions=1
  IMAPve_d_TCU_Select_ATMode : Outport  Port=109  OutDataTypeStr=uint16  PortDimensions=1
  IMAPve_d_EMS_Engine_Status : Outport  Port=110  OutDataTypeStr=uint16  PortDimensions=1
  IMAPve_d_EMS_Gearbox_CtlAvail : Outport  Port=111  OutDataTypeStr=uint16  PortDimensions=1
  IMAPve_d_ESC_Brake_Failsafe : Outport  Port=112  OutDataTypeStr=uint16  PortDimensions=1
  IMAPve_d_ESC_AEB_Available : Outport  Port=113  OutDataTypeStr=uint16  PortDimensions=1
  IMAPve_d_ESC_AEB_Active : Outport  Port=114  OutDataTypeStr=uint16  PortDimensions=1
  IMAPve_d_ESC_ACC_Available : Outport  Port=115  OutDataTypeStr=uint16  PortDimensions=1
  IMAPve_d_ESC_ACC_Active : Outport  Port=116  OutDataTypeStr=uint16  PortDimensions=1
  IMAPve_d_EMS_ACC_Effective : Outport  Port=117  OutDataTypeStr=uint16  PortDimensions=1
  IMAPve_d_BCM_FrontWiper_State : Outport  Port=118  OutDataTypeStr=uint16  PortDimensions=1
  IMAPve_d_BCM_CHMSL_Status : Outport  Port=119  OutDataTypeStr=uint16  PortDimensions=1
  IMAPve_d_BCM_BrakeLamp_State : Outport  Port=120  OutDataTypeStr=uint16  PortDimensions=1
  IMAPve_d_ACU_Passenger_Belt : Outport  Port=121  OutDataTypeStr=uint16  PortDimensions=1
  IMAPve_d_EMS_ACC_CtlAvail : Outport  Port=122  OutDataTypeStr=uint16  PortDimensions=1
  IMAPve_d_EMS_ACC_Inhibited : Outport  Port=123  OutDataTypeStr=uint16  PortDimensions=1
  IMAPve_d_EMS_Brake_Pedal : Outport  Port=124  OutDataTypeStr=uint16  PortDimensions=1
  IMAPve_d_BCM_LowBeam_State : Outport  Port=125  OutDataTypeStr=uint16  PortDimensions=1
  IMAPve_d_BCM_HighBeam_State : Outport  Port=126  OutDataTypeStr=uint16  PortDimensions=1
  IMAPve_d_EPB_Status : Outport  Port=127  OutDataTypeStr=uint16  PortDimensions=1
  IMAPve_d_EPB_Display_Req : Outport  Port=128  OutDataTypeStr=uint16  PortDimensions=1
  IMAPve_d_EPB_Warn_Req : Outport  Port=129  OutDataTypeStr=uint16  PortDimensions=1
  IMAPve_d_EPB_Switch_State : Outport  Port=130  OutDataTypeStr=uint16  PortDimensions=1
  IMAPve_d_EPB_Switch_Valid : Outport  Port=131  OutDataTypeStr=uint16  PortDimensions=1
  IMAPve_d_ESC_Drive_Direction : Outport  Port=132  OutDataTypeStr=uint16  PortDimensions=1
  IMAPve_d_ESC_Hold_State : Outport  Port=133  OutDataTypeStr=uint16  PortDimensions=1
  IMAPve_d_EPS_Steer_Hold_State : Outport  Port=134  OutDataTypeStr=uint16  PortDimensions=1
  IMAPve_d_EPS_Warning_State : Outport  Port=135  OutDataTypeStr=uint16  PortDimensions=1
  IMAPve_g_EPS_PowerCon : Outport  Port=136  OutDataTypeStr=single  PortDimensions=1
  IMAPve_d_ESC_EBD_AlarmSig : Outport  Port=137  OutDataTypeStr=uint16  PortDimensions=1
  IMAPve_d_ESC_AVH_Status : Outport  Port=138  OutDataTypeStr=uint16  PortDimensions=1
  IMAPve_g_BCM_Battery_Voltage : Outport  Port=139  OutDataTypeStr=single  PortDimensions=1
  IMAPve_d_TBOX_LocalTimeY : Outport  Port=140  OutDataTypeStr=uint16  PortDimensions=1
  IMAPve_d_TBOX_LocalTimeM : Outport  Port=141  OutDataTypeStr=uint16  PortDimensions=1
  IMAPve_d_TBOX_LocalTimeD : Outport  Port=142  OutDataTypeStr=uint16  PortDimensions=1
  IMAPve_d_TBOX_LocalTimeH : Outport  Port=143  OutDataTypeStr=uint16  PortDimensions=1
  IMAPve_d_TBOX_LocalTimeMin : Outport  Port=144  OutDataTypeStr=uint16  PortDimensions=1
  IMAPve_d_TBOX_LocalTimeS : Outport  Port=145  OutDataTypeStr=uint16  PortDimensions=1
  IMAPve_d_TBOX_LocalTime_Valid : Outport  Port=146  OutDataTypeStr=uint16  PortDimensions=1
  IMAPve_d_Radar_State : Outport  Port=147  OutDataTypeStr=uint16  PortDimensions=1
  IMAPve_d_Time_System_Clock : Outport  Port=148  OutDataTypeStr=uint16  PortDimensions=1
  IMAPve_g_GW_IC_Odometer : Outport  Port=149  OutDataTypeStr=uint32  PortDimensions=1
  IMAPve_d_Outside_Temp : Outport  Port=150  OutDataTypeStr=uint16  PortDimensions=1
  IMAPve_d_ORI_CIPV_ID : Outport  Port=151  OutDataTypeStr=uint16  PortDimensions=1
  IMAPve_d_ORI_Obj_Num : Outport  Port=152  OutDataTypeStr=uint16  PortDimensions=1
  IMAPva_d_ORI_Obj_Class : Outport  Port=153  OutDataTypeStr=uint16  PortDimensions=20
  IMAPva_g_ORI_Obj_RelVel : Outport  Port=154  OutDataTypeStr=single  PortDimensions=20
  IMAPva_g_ORI_Obj_LongDis : Outport  Port=155  OutDataTypeStr=single  PortDimensions=20
  IMAPva_g_ORI_Obj_LAngle : Outport  Port=156  OutDataTypeStr=single  PortDimensions=20
  IMAPva_g_ORI_Obj_RAngle : Outport  Port=157  OutDataTypeStr=single  PortDimensions=20
  IMAPva_g_ORI_Obj_Width : Outport  Port=158  OutDataTypeStr=single  PortDimensions=20
  IMAPva_d_ORI_Obj_ID : Outport  Port=159  OutDataTypeStr=uint16  PortDimensions=20
  IMAPve_g_ORI_L0_C3 : Outport  Port=160  OutDataTypeStr=single  PortDimensions=1
  IMAPve_g_ORI_L0_C2 : Outport  Port=161  OutDataTypeStr=single  PortDimensions=1
  IMAPve_g_ORI_L0_C1 : Outport  Port=162  OutDataTypeStr=single  PortDimensions=1
  IMAPve_g_ORI_L0_C0 : Outport  Port=163  OutDataTypeStr=single  PortDimensions=1
  IMAPve_d_ORI_L0_Type : Outport  Port=164  OutDataTypeStr=uint16  PortDimensions=1
  IMAPve_g_ORI_L0_VR : Outport  Port=165  OutDataTypeStr=single  PortDimensions=1
  IMAPve_g_ORI_L0_W : Outport  Port=166  OutDataTypeStr=single  PortDimensions=1
  IMAPve_g_ORI_L1_C3 : Outport  Port=167  OutDataTypeStr=single  PortDimensions=1
  IMAPve_g_ORI_L1_C2 : Outport  Port=168  OutDataTypeStr=single  PortDimensions=1
  IMAPve_g_ORI_L1_C1 : Outport  Port=169  OutDataTypeStr=single  PortDimensions=1
  IMAPve_g_ORI_L1_C0 : Outport  Port=170  OutDataTypeStr=single  PortDimensions=1
  IMAPve_d_ORI_L1_Type : Outport  Port=171  OutDataTypeStr=uint16  PortDimensions=1
  IMAPve_g_ORI_L1_VR : Outport  Port=172  OutDataTypeStr=single  PortDimensions=1
  IMAPve_g_ORI_L1_W : Outport  Port=173  OutDataTypeStr=single  PortDimensions=1
  IMAPve_g_ORI_R0_C3 : Outport  Port=174  OutDataTypeStr=single  PortDimensions=1
  IMAPve_g_ORI_R0_C2 : Outport  Port=175  OutDataTypeStr=single  PortDimensions=1
  IMAPve_g_ORI_R0_C1 : Outport  Port=176  OutDataTypeStr=single  PortDimensions=1
  IMAPve_g_ORI_R0_C0 : Outport  Port=177  OutDataTypeStr=single  PortDimensions=1
  IMAPve_d_ORI_R0_LT : Outport  Port=178  OutDataTypeStr=uint16  PortDimensions=1
  IMAPve_g_ORI_R0_VR : Outport  Port=179  OutDataTypeStr=single  PortDimensions=1
  IMAPve_g_ORI_R0_W : Outport  Port=180  OutDataTypeStr=single  PortDimensions=1
  IMAPve_g_ORI_R1_C3 : Outport  Port=181  OutDataTypeStr=single  PortDimensions=1
  IMAPve_g_ORI_R1_C2 : Outport  Port=182  OutDataTypeStr=single  PortDimensions=1
  IMAPve_g_ORI_R1_C1 : Outport  Port=183  OutDataTypeStr=single  PortDimensions=1
  IMAPve_g_ORI_R1_C0 : Outport  Port=184  OutDataTypeStr=single  PortDimensions=1
  IMAPve_d_ORI_R1_LT : Outport  Port=185  OutDataTypeStr=uint16  PortDimensions=1
  IMAPve_g_ORI_R1_VR : Outport  Port=186  OutDataTypeStr=single  PortDimensions=1
  IMAPve_g_ORI_R1_W : Outport  Port=187  OutDataTypeStr=single  PortDimensions=1
  IMAPve_d_Sensor_Status : Outport  Port=188  OutDataTypeStr=uint16  PortDimensions=1
  IMAPve_d_LF_Radar_Status : Outport  Port=189  OutDataTypeStr=uint16  PortDimensions=1
  IMAPve_d_RF_Radar_Status : Outport  Port=190  OutDataTypeStr=uint16  PortDimensions=1
  IMAPve_d_LR_Radar_Status : Outport  Port=191  OutDataTypeStr=uint16  PortDimensions=1
  IMAPve_d_RR_Radar_Status : Outport  Port=192  OutDataTypeStr=uint16  PortDimensions=1
  IMAPve_d_Fusion_Status : Outport  Port=193  OutDataTypeStr=uint16  PortDimensions=1
  IMAPve_d_Fusion_Time_Stamp : Outport  Port=194  OutDataTypeStr=uint16  PortDimensions=1
  IMAPve_d_obj_Num : Outport  Port=195  OutDataTypeStr=uint16  PortDimensions=1
  IMAPva_d_obj_id : Outport  Port=196  OutDataTypeStr=uint16  PortDimensions=40
  IMAPva_g_obj_pos_x : Outport  Port=197  OutDataTypeStr=single  PortDimensions=40
  IMAPva_g_obj_pos_y : Outport  Port=198  OutDataTypeStr=single  PortDimensions=40
  IMAPva_g_obj_vel_x : Outport  Port=199  OutDataTypeStr=single  PortDimensions=40
  IMAPva_g_obj_vel_y : Outport  Port=200  OutDataTypeStr=single  PortDimensions=40
  IMAPva_g_obj_acc_x : Outport  Port=201  OutDataTypeStr=single  PortDimensions=40
  IMAPva_g_obj_acc_y : Outport  Port=202  OutDataTypeStr=single  PortDimensions=40
  IMAPva_g_obj_pos_var_x : Outport  Port=203  OutDataTypeStr=single  PortDimensions=40
  IMAPva_g_obj_pos_var_y : Outport  Port=204  OutDataTypeStr=single  PortDimensions=40
  IMAPva_g_obj_pos_var_xy : Outport  Port=205  OutDataTypeStr=single  PortDimensions=40
  IMAPva_g_obj_width : Outport  Port=206  OutDataTypeStr=single  PortDimensions=40
  IMAPva_g_obj_length : Outport  Port=207  OutDataTypeStr=single  PortDimensions=40
  IMAPva_d_obj_class : Outport  Port=208  OutDataTypeStr=uint16  PortDimensions=40
  IMAPva_d_obj_lane : Outport  Port=209  OutDataTypeStr=uint16  PortDimensions=40
  IMAPva_d_obj_status : Outport  Port=210  OutDataTypeStr=uint16  PortDimensions=40
  IMAPva_d_obj_age : Outport  Port=211  OutDataTypeStr=uint16  PortDimensions=40
  IMAPva_d_obj_TurnLight : Outport  Port=212  OutDataTypeStr=uint16  PortDimensions=40
  IMAPva_d_obj_BrakeLight : Outport  Port=213  OutDataTypeStr=uint16  PortDimensions=40
  IMAPva_d_obj_MotionStatus : Outport  Port=214  OutDataTypeStr=uint16  PortDimensions=40
  IMAPve_d_Road_Type : Outport  Port=215  OutDataTypeStr=uint16  PortDimensions=1
  IMAPve_g_L0_C0 : Outport  Port=216  OutDataTypeStr=single  PortDimensions=1
  IMAPve_g_L0_C1 : Outport  Port=217  OutDataTypeStr=single  PortDimensions=1
  IMAPve_g_L0_C2 : Outport  Port=218  OutDataTypeStr=single  PortDimensions=1
  IMAPve_g_L0_C3 : Outport  Port=219  OutDataTypeStr=single  PortDimensions=1
  IMAPve_g_L0_VR : Outport  Port=220  OutDataTypeStr=single  PortDimensions=1
  IMAPve_d_L0_Q : Outport  Port=221  OutDataTypeStr=uint16  PortDimensions=1
  IMAPve_d_L0_Type : Outport  Port=222  OutDataTypeStr=uint16  PortDimensions=1
  IMAPve_g_L0_W : Outport  Port=223  OutDataTypeStr=single  PortDimensions=1
  IMAPve_g_R0_C0 : Outport  Port=224  OutDataTypeStr=single  PortDimensions=1
  IMAPve_g_R0_C1 : Outport  Port=225  OutDataTypeStr=single  PortDimensions=1
  IMAPve_g_R0_C2 : Outport  Port=226  OutDataTypeStr=single  PortDimensions=1
  IMAPve_g_R0_C3 : Outport  Port=227  OutDataTypeStr=single  PortDimensions=1
  IMAPve_g_R0_VR : Outport  Port=228  OutDataTypeStr=single  PortDimensions=1
  IMAPve_d_R0_Q : Outport  Port=229  OutDataTypeStr=uint16  PortDimensions=1
  IMAPve_d_R0_Type : Outport  Port=230  OutDataTypeStr=uint16  PortDimensions=1
  IMAPve_g_R0_W : Outport  Port=231  OutDataTypeStr=single  PortDimensions=1
  IMAPve_g_L1_C0 : Outport  Port=232  OutDataTypeStr=single  PortDimensions=1
  IMAPve_g_L1_C1 : Outport  Port=233  OutDataTypeStr=single  PortDimensions=1
  IMAPve_g_L1_C2 : Outport  Port=234  OutDataTypeStr=single  PortDimensions=1
  IMAPve_g_L1_C3 : Outport  Port=235  OutDataTypeStr=single  PortDimensions=1
  IMAPve_g_L1_VR : Outport  Port=236  OutDataTypeStr=single  PortDimensions=1
  IMAPve_d_L1_Q : Outport  Port=237  OutDataTypeStr=uint16  PortDimensions=1
  IMAPve_d_L1_Type : Outport  Port=238  OutDataTypeStr=uint16  PortDimensions=1
  IMAPve_g_L1_W : Outport  Port=239  OutDataTypeStr=single  PortDimensions=1
  IMAPve_g_R1_C0 : Outport  Port=240  OutDataTypeStr=single  PortDimensions=1
  IMAPve_g_R1_C1 : Outport  Port=241  OutDataTypeStr=single  PortDimensions=1
  IMAPve_g_R1_C2 : Outport  Port=242  OutDataTypeStr=single  PortDimensions=1
  IMAPve_g_R1_C3 : Outport  Port=243  OutDataTypeStr=single  PortDimensions=1
  IMAPve_g_R1_VR : Outport  Port=244  OutDataTypeStr=single  PortDimensions=1
  IMAPve_d_R1_Q : Outport  Port=245  OutDataTypeStr=uint16  PortDimensions=1
  IMAPve_d_R1_Type : Outport  Port=246  OutDataTypeStr=uint16  PortDimensions=1
  IMAPve_g_R1_W : Outport  Port=247  OutDataTypeStr=single  PortDimensions=1
  IMAPve_g_L0_C0_Back : Outport  Port=248  OutDataTypeStr=single  PortDimensions=1
  IMAPve_g_L0_C1_Back : Outport  Port=249  OutDataTypeStr=single  PortDimensions=1
  IMAPve_g_L0_C2_Back : Outport  Port=250  OutDataTypeStr=single  PortDimensions=1
  IMAPve_g_L0_C3_Back : Outport  Port=251  OutDataTypeStr=single  PortDimensions=1
  IMAPve_g_L0_Range_Back : Outport  Port=252  OutDataTypeStr=single  PortDimensions=1
  IMAPve_g_R0_C0_Back : Outport  Port=253  OutDataTypeStr=single  PortDimensions=1
  IMAPve_g_R0_C1_Back : Outport  Port=254  OutDataTypeStr=single  PortDimensions=1
  IMAPve_g_R0_C2_Back : Outport  Port=255  OutDataTypeStr=single  PortDimensions=1
  IMAPve_g_R0_C3_Back : Outport  Port=256  OutDataTypeStr=single  PortDimensions=1
  IMAPve_g_R0_Range_Back : Outport  Port=257  OutDataTypeStr=single  PortDimensions=1
  IMAPve_g_L1_C0_Back : Outport  Port=258  OutDataTypeStr=single  PortDimensions=1
  IMAPve_g_L1_C1_Back : Outport  Port=259  OutDataTypeStr=single  PortDimensions=1
  IMAPve_g_L1_C2_Back : Outport  Port=260  OutDataTypeStr=single  PortDimensions=1
  IMAPve_g_L1_C3_Back : Outport  Port=261  OutDataTypeStr=single  PortDimensions=1
  IMAPve_g_L1_Range_Back : Outport  Port=262  OutDataTypeStr=single  PortDimensions=1
  IMAPve_g_R1_C0_Back : Outport  Port=263  OutDataTypeStr=single  PortDimensions=1
  IMAPve_g_R1_C1_Back : Outport  Port=264  OutDataTypeStr=single  PortDimensions=1
  IMAPve_g_R1_C2_Back : Outport  Port=265  OutDataTypeStr=single  PortDimensions=1
  IMAPve_g_R1_C3_Back : Outport  Port=266  OutDataTypeStr=single  PortDimensions=1
  IMAPve_g_R1_Range_Back : Outport  Port=267  OutDataTypeStr=single  PortDimensions=1
  IMAPve_g_Lrg_C0_BACK : Outport  Port=268  OutDataTypeStr=single
  IMAPve_g_Lrg_C1_BACK : Outport  Port=269  OutDataTypeStr=single
  IMAPve_g_Lrg_C2_BACK : Outport  Port=270  OutDataTypeStr=single
  IMAPve_g_Lrg_C3_BACK : Outport  Port=271  OutDataTypeStr=single
  IMAPve_g_Lrg_VR_Start_BACK : Outport  Port=272  OutDataTypeStr=single
  IMAPve_g_Lrg_VR_End_BACK : Outport  Port=273  OutDataTypeStr=single
  IMAPve_d_Lrg_Q_BACK : Outport  Port=274  OutDataTypeStr=uint16
  IMAPve_d_Lrg_TYPE_BACK : Outport  Port=275  OutDataTypeStr=uint16
  IMAPve_g_Rrg_C0_BACK : Outport  Port=276  OutDataTypeStr=single
  IMAPve_g_Rrg_C1_BACK : Outport  Port=277  OutDataTypeStr=single
  IMAPve_g_Rrg_C2_BACK : Outport  Port=278  OutDataTypeStr=single
  IMAPve_g_Rrg_C3_BACK : Outport  Port=279  OutDataTypeStr=single
  IMAPve_g_Rrg_VR_Start_BACK : Outport  Port=280  OutDataTypeStr=single
  IMAPve_g_Rrg_VR_End_BACK : Outport  Port=281  OutDataTypeStr=single
  IMAPve_d_Rrg_Q_BACK : Outport  Port=282  OutDataTypeStr=uint16
  IMAPve_d_Rrg_TYPE_BACK : Outport  Port=283  OutDataTypeStr=uint16
  IMAPve_d_Sign_ISA_Value : Outport  Port=284  OutDataTypeStr=uint16  PortDimensions=1
  IMAPve_d_ISA_Popup_Message : Outport  Port=285  OutDataTypeStr=uint16
  IMAPve_d_ISA_Sign_Type : Outport  Port=286  OutDataTypeStr=uint16
  IMAPve_d_ISA_Status : Outport  Port=287  OutDataTypeStr=uint16
  IMAPve_d_TSR_Sign_Type : Outport  Port=288  OutDataTypeStr=uint16  PortDimensions=1
  IMAPve_g_Camera_Signal_Fault : Outport  Port=289  OutDataTypeStr=single  PortDimensions=1
  IMAPve_d_Camera_State : Outport  Port=290  OutDataTypeStr=uint16  PortDimensions=1
  IMAPve_d_Radar_FaultBitSetting_Signal : Outport  Port=291
  IMAPve_d_Camera_Status : Outport  Port=292  OutDataTypeStr=uint16  PortDimensions=1
  IMAPve_d_ESC_FLW_Direction : Outport  Port=293  OutDataTypeStr=uint16
  IMAPve_d_ESC_FRW_Direction : Outport  Port=294  OutDataTypeStr=uint16
  IMAPve_d_ESC_TCS_ErrorStatus : Outport  Port=295  OutDataTypeStr=uint16
  IMAPve_d_ESC_RLW_Direction : Outport  Port=296  OutDataTypeStr=uint16
  IMAPve_d_ESC_RRW_Direction : Outport  Port=297  OutDataTypeStr=uint16
  IMAPve_d_ESC_EPB_ErrorStatus : Outport  Port=298  OutDataTypeStr=uint16
  IMAPve_d_EPS_SteeringAngle_Flag : Outport  Port=299  OutDataTypeStr=uint16
  IMAPve_g_EPS_SteeringAngle : Outport  Port=300  OutDataTypeStr=single
  IMAPve_d_EPS_Driver_Override : Outport  Port=301  OutDataTypeStr=uint16
  IMAPve_d_EPS_Driver_Active_ESA : Outport  Port=302  OutDataTypeStr=uint16
  IMAPve_d_EPS_ESA_State : Outport  Port=303  OutDataTypeStr=uint16
  IMAPve_d_ACU_RearLeft_Belt : Outport  Port=304  OutDataTypeStr=uint16
  IMAPve_d_ACU_RearMiddle_Belt : Outport  Port=305  OutDataTypeStr=uint16
  IMAPve_d_ACU_RearRight_Belt : Outport  Port=306  OutDataTypeStr=uint16
  IMAPve_d_EMS_PowertrainCtl_State : Outport  Port=307  OutDataTypeStr=uint16
  IMAPve_d_TCU_TCU_Available : Outport  Port=308  OutDataTypeStr=uint16
  IMAPve_d_BCM_LeftTurn_Switch : Outport  Port=309  OutDataTypeStr=uint16
  IMAPve_d_BCM_RightTurn_Switch : Outport  Port=310  OutDataTypeStr=uint16
  IMAPve_d_BCM_FrontWiper_Switch : Outport  Port=311  OutDataTypeStr=uint16
  IMAPve_d_BCM_IHBC_Enabled : Outport  Port=312  OutDataTypeStr=uint16
  IMAPve_d_MP5_Work_State : Outport  Port=313  OutDataTypeStr=uint16
  IMAPve_d_MP5_APA_ModeSelect : Outport  Port=314  OutDataTypeStr=uint16
  IMAPve_d_MP5_LanguageSet : Outport  Port=315  OutDataTypeStr=uint16
  IMAPve_d_MP5_UPA_Switch : Outport  Port=316  OutDataTypeStr=uint16
  IMAPve_d_MP5_FLK_Activation : Outport  Port=317  OutDataTypeStr=uint16
  IMAPve_d_MP5_AutoPilot_Switch : Outport  Port=318  OutDataTypeStr=uint16
  IMAPve_d_MP5_DMS_MessageType : Outport  Port=319  OutDataTypeStr=uint16
  IMAPve_d_MP5_DMS_SystemEnable : Outport  Port=320  OutDataTypeStr=uint16
  IMAPve_d_MP5_DMS_DelUserNum : Outport  Port=321  OutDataTypeStr=uint16
  IMAPve_d_MP5_DMS_Sensity : Outport  Port=322  OutDataTypeStr=uint16
  IMAPve_d_MP5_DMS_EyeFatigue : Outport  Port=323  OutDataTypeStr=uint16
  IMAPve_d_MP5_DMS_LongtimeDrive : Outport  Port=324  OutDataTypeStr=uint16
  IMAPve_d_MP5_DMS_SideView : Outport  Port=325  OutDataTypeStr=uint16
  IMAPve_d_MP5_DMS_UsingPhone : Outport  Port=326  OutDataTypeStr=uint16
  IMAPve_d_MP5_DMS_Smoking : Outport  Port=327  OutDataTypeStr=uint16
  IMAPve_d_MP5_DMS_DrinkWater : Outport  Port=328  OutDataTypeStr=uint16
  IMAPve_d_MP5_DMS_UserAccount : Outport  Port=329  OutDataTypeStr=uint16
  IMAPve_g_ESC_BrkWhlCylinder_Pressure : Outport  Port=330  OutDataTypeStr=single
  IMAPva_d_ORI_Obj_TimeStamp : Outport  Port=331  OutDataTypeStr=uint16  PortDimensions=20
  IMAPve_d_ORI_FS_OutOfCalib : Outport  Port=332  OutDataTypeStr=uint16
  IMAPve_d_ORI_FS_Rain : Outport  Port=333  OutDataTypeStr=uint16
  IMAPve_d_ORI_FS_Fog : Outport  Port=334  OutDataTypeStr=uint16
  IMAPve_d_ORI_FS_Splashes0 : Outport  Port=335  OutDataTypeStr=uint16
  IMAPve_d_ORI_FS_SunRay0 : Outport  Port=336  OutDataTypeStr=uint16
  IMAPve_d_ORI_FS_LowSun0 : Outport  Port=337  OutDataTypeStr=uint16
  IMAPve_d_ORI_FS_BlurImage0 : Outport  Port=338  OutDataTypeStr=uint16
  IMAPve_d_ORI_FS_PartialBlockage0 : Outport  Port=339  OutDataTypeStr=uint16
  IMAPve_d_ORI_FS_FullBlockage0 : Outport  Port=340  OutDataTypeStr=uint16
  IMAPve_d_ORI_FS_FrozenWindshield0 : Outport  Port=341  OutDataTypeStr=uint16
  IMAPve_d_ORI_FS_OutOfFocus0 : Outport  Port=342  OutDataTypeStr=uint16
  IMAPva_g_ORI_Obj_AbsAx : Outport  Port=343  OutDataTypeStr=single  PortDimensions=20
  IMAPva_g_ORI_Obj_AbsAy : Outport  Port=344  OutDataTypeStr=single  PortDimensions=20
  IMAPva_g_ORI_Obj_TTIPCStdDev : Outport  Port=345  OutDataTypeStr=single  PortDimensions=20
  IMAPva_g_ORI_Obj_RelVely : Outport  Port=346  OutDataTypeStr=single  PortDimensions=20
  IMAPva_g_ORI_Obj_LateralDis : Outport  Port=347  OutDataTypeStr=single  PortDimensions=20
  IMAPva_g_ORI_Obj_AbsAxStdDev : Outport  Port=348  OutDataTypeStr=single  PortDimensions=20
  IMAPva_g_ORI_Obj_AbsAyStdDev : Outport  Port=349  OutDataTypeStr=single  PortDimensions=20
  IMAPva_g_ORI_Obj_RelVelStdDev : Outport  Port=350  OutDataTypeStr=single  PortDimensions=20
  IMAPva_g_ORI_Obj_RelVelyStdDev : Outport  Port=351  OutDataTypeStr=single  PortDimensions=20
  IMAPva_g_ORI_Obj_LongDisStdDev : Outport  Port=352  OutDataTypeStr=single  PortDimensions=20
  IMAPva_g_ORI_Obj_LateralDisStdDev : Outport  Port=353  OutDataTypeStr=single  PortDimensions=20
  IMAPva_d_ORI_Obj_RelVelValid : Outport  Port=354  OutDataTypeStr=uint16  PortDimensions=20
  IMAPva_d_ORI_Obj_RelVelyValid : Outport  Port=355  OutDataTypeStr=uint16  PortDimensions=20
  IMAPva_d_ORI_Obj_RelVelStdDevValid : Outport  Port=356  OutDataTypeStr=uint16  PortDimensions=20
  IMAPva_d_ORI_Obj_RelVelyStdDevValid : Outport  Port=357  OutDataTypeStr=uint16  PortDimensions=20
  IMAPva_g_ORI_Obj_ExistProb : Outport  Port=358  OutDataTypeStr=single  PortDimensions=20
  IMAPva_g_ORI_Obj_ClassProb : Outport  Port=359  OutDataTypeStr=single  PortDimensions=20
  IMAPva_g_ORI_Obj_Height : Outport  Port=360  OutDataTypeStr=single  PortDimensions=20
  IMAPva_g_ORI_Obj_LengthStdDev : Outport  Port=361  OutDataTypeStr=single  PortDimensions=20
  IMAPva_g_ORI_Obj_WidthStdDev : Outport  Port=362  OutDataTypeStr=single  PortDimensions=20
  IMAPva_g_ORI_Obj_HeightStdDev : Outport  Port=363  OutDataTypeStr=single  PortDimensions=20
  IMAPva_g_ORI_Obj_3DAngle : Outport  Port=364  OutDataTypeStr=single  PortDimensions=20
  IMAPva_g_ORI_Obj_LAngleStdDev : Outport  Port=365  OutDataTypeStr=single  PortDimensions=20
  IMAPva_g_ORI_Obj_RAngleStdDev : Outport  Port=366  OutDataTypeStr=single  PortDimensions=20
  IMAPva_g_ORI_Obj_3DAngleStdDev : Outport  Port=367  OutDataTypeStr=single  PortDimensions=20
  IMAPva_g_ORI_Obj_AngleRate : Outport  Port=368  OutDataTypeStr=single  PortDimensions=20
  IMAPva_g_ORI_Obj_AngleRateStdDev : Outport  Port=369  OutDataTypeStr=single  PortDimensions=20
  IMAPva_g_ORI_Obj_PhiBottom : Outport  Port=370  OutDataTypeStr=single  PortDimensions=20
  IMAPva_g_ORI_Obj_PhiBottomStdDev : Outport  Port=371  OutDataTypeStr=single  PortDimensions=20
  IMAPva_d_ORI_Obj_Measured : Outport  Port=372  OutDataTypeStr=uint16  PortDimensions=20
  IMAPva_g_ORI_Obj_Heading : Outport  Port=373  OutDataTypeStr=single  PortDimensions=20
  IMAPva_g_ORI_Obj_HeadingStdDev : Outport  Port=374  OutDataTypeStr=single  PortDimensions=20
  IMAPva_d_ORI_Obj_HeadOrientation : Outport  Port=375  OutDataTypeStr=uint16  PortDimensions=20
  IMAPva_g_ORI_Obj_TTIPC : Outport  Port=376  OutDataTypeStr=single  PortDimensions=20
  IMAPva_d_ORI_Obj_DirectionIndicator : Outport  Port=377  OutDataTypeStr=uint16  PortDimensions=20
  IMAPva_d_ORI_Obj_BrakeLight : Outport  Port=378  OutDataTypeStr=uint16  PortDimensions=20
  IMAPve_d_ORI_L0_ID : Outport  Port=379  OutDataTypeStr=uint16
  IMAPve_g_ORI_L0_ExistProb : Outport  Port=380  OutDataTypeStr=single
  IMAPve_g_ORI_L0_DxStart : Outport  Port=381  OutDataTypeStr=single
  IMAPve_d_ORI_L0_ColorClass : Outport  Port=382  OutDataTypeStr=uint16
  IMAPve_d_ORI_L0_MeasureType : Outport  Port=383  OutDataTypeStr=uint16
  IMAPve_g_ORI_L0_TypeConf : Outport  Port=384  OutDataTypeStr=single
  IMAPve_d_ORI_R0_ID : Outport  Port=385  OutDataTypeStr=uint16
  IMAPve_g_ORI_R0_ExistProb : Outport  Port=386  OutDataTypeStr=single
  IMAPve_g_ORI_R0_Dxstart : Outport  Port=387  OutDataTypeStr=single
  IMAPve_d_ORI_R0_ColorClass : Outport  Port=388  OutDataTypeStr=uint16
  IMAPve_d_ORI_R0_MeasureType : Outport  Port=389  OutDataTypeStr=uint16
  IMAPve_g_ORI_R0_TypeConf : Outport  Port=390  OutDataTypeStr=single
  IMAPve_d_ORI_L1_ID : Outport  Port=391  OutDataTypeStr=uint16
  IMAPve_g_ORI_L1_ExistProb : Outport  Port=392  OutDataTypeStr=single
  IMAPve_g_ORI_L1_Dxstart : Outport  Port=393  OutDataTypeStr=single
  IMAPve_d_ORI_L1_ColorClass : Outport  Port=394  OutDataTypeStr=uint16
  IMAPve_d_ORI_L1_MeasureType : Outport  Port=395  OutDataTypeStr=uint16
  IMAPve_g_ORI_L1_TypeConf : Outport  Port=396  OutDataTypeStr=single
  IMAPve_d_ORI_R1_ID : Outport  Port=397  OutDataTypeStr=uint16
  IMAPve_g_ORI_R1_ExistProb : Outport  Port=398  OutDataTypeStr=single
  IMAPve_g_ORI_R1_Dxstart : Outport  Port=399  OutDataTypeStr=single
  IMAPve_d_ORI_R1_ColorClass : Outport  Port=400  OutDataTypeStr=uint16
  IMAPve_d_ORI_R1_MeasureType : Outport  Port=401  OutDataTypeStr=uint16
  IMAPve_g_ORI_R1_TypeConf : Outport  Port=402  OutDataTypeStr=single
  IMAPve_d_ORI_RoadedgeL0_ID : Outport  Port=403  OutDataTypeStr=uint16
  IMAPve_g_ORI_RoadedgeL0_ExistProb : Outport  Port=404  OutDataTypeStr=single
  IMAPve_g_ORI_RoadedgeL0_DxStart : Outport  Port=405  OutDataTypeStr=single
  IMAPve_g_ORI_RoadedgeL0_DxEnd : Outport  Port=406  OutDataTypeStr=single
  IMAPve_g_ORI_RoadedgeL0_C1 : Outport  Port=407  OutDataTypeStr=single
  IMAPve_g_ORI_RoadedgeL0_C0 : Outport  Port=408  OutDataTypeStr=single
  IMAPve_g_ORI_RoadedgeL0_C3 : Outport  Port=409  OutDataTypeStr=single
  IMAPve_g_ORI_RoadedgeL0_C2 : Outport  Port=410  OutDataTypeStr=single
  IMAPve_d_ORI_RoadedgeL0_MeasureType : Outport  Port=411  OutDataTypeStr=uint16
  IMAPve_d_ORI_RoadedgeL0_Type : Outport  Port=412  OutDataTypeStr=uint16
  IMAPve_d_ORI_RoadedgeR0_ID : Outport  Port=413  OutDataTypeStr=uint16
  IMAPve_g_ORI_RoadedgeR0_ExistProb : Outport  Port=414  OutDataTypeStr=single
  IMAPve_g_ORI_RoadedgeR0_DxStart : Outport  Port=415  OutDataTypeStr=single
  IMAPve_g_ORI_RoadedgeR0_DxEnd : Outport  Port=416  OutDataTypeStr=single
  IMAPve_g_ORI_RoadedgeR0_C1 : Outport  Port=417  OutDataTypeStr=single
  IMAPve_g_ORI_RoadedgeR0_C0 : Outport  Port=418  OutDataTypeStr=single
  IMAPve_g_ORI_RoadedgeR0_C3 : Outport  Port=419  OutDataTypeStr=single
  IMAPve_g_ORI_RoadedgeR0_C2 : Outport  Port=420  OutDataTypeStr=single
  IMAPve_d_ORI_RoadedgeR0_MeasureType : Outport  Port=421  OutDataTypeStr=uint16
  IMAPve_d_ORI_RoadedgeR0_Type : Outport  Port=422  OutDataTypeStr=uint16
  IMAPve_d_APA_AutoPark_WorkSt : Outport  Port=423  OutDataTypeStr=uint16
  IMAPve_g_ob020H_100 : Outport  Port=424  OutDataTypeStr=uint32
  IMAPve_g_ob020L_100 : Outport  Port=425  OutDataTypeStr=uint32
  wires:
  SWINve_y_T_box_RemoteHazardReq/1 -> IMAP_Module/41(SWINve_y_T_box_RemoteHazardReq)
  SWINve_y_MP5_HazardLampCtrlReq/1 -> IMAP_Module/40(SWINve_y_MP5_HazardLampCtrlReq)
  SWINve_y_BCM_HazardSwitchrSt/1 -> IMAP_Module/39(SWINve_y_BCM_HazardSwitchrSt)
  IMAP_Module/283(IMAPve_d_Rrg_TYPE_BACK) -> IMAPve_d_Rrg_TYPE_BACK/1
  IMAP_Module/282(IMAPve_d_Rrg_Q_BACK) -> IMAPve_d_Rrg_Q_BACK/1
  IMAP_Module/281(IMAPve_g_Rrg_VR_End_BACK) -> IMAPve_g_Rrg_VR_End_BACK/1
  IMAP_Module/280(IMAPve_g_Rrg_VR_Start_BACK) -> IMAPve_g_Rrg_VR_Start_BACK/1
  IMAP_Module/279(IMAPve_g_Rrg_C3_BACK) -> IMAPve_g_Rrg_C3_BACK/1
  IMAP_Module/278(IMAPve_g_Rrg_C2_BACK) -> IMAPve_g_Rrg_C2_BACK/1
  IMAP_Module/277(IMAPve_g_Rrg_C1_BACK) -> IMAPve_g_Rrg_C1_BACK/1
  IMAP_Module/276(IMAPve_g_Rrg_C0_BACK) -> IMAPve_g_Rrg_C0_BACK/1
  IMAP_Module/275(IMAPve_d_Lrg_TYPE_BACK) -> IMAPve_d_Lrg_TYPE_BACK/1
  IMAP_Module/274(IMAPve_d_Lrg_Q_BACK) -> IMAPve_d_Lrg_Q_BACK/1
  IMAP_Module/273(IMAPve_g_Lrg_VR_End_BACK) -> IMAPve_g_Lrg_VR_End_BACK/1
  IMAP_Module/272(IMAPve_g_Lrg_VR_Start_BACK) -> IMAPve_g_Lrg_VR_Start_BACK/1
  IMAP_Module/271(IMAPve_g_Lrg_C3_BACK) -> IMAPve_g_Lrg_C3_BACK/1
  IMAP_Module/270(IMAPve_g_Lrg_C2_BACK) -> IMAPve_g_Lrg_C2_BACK/1
  IMAP_Module/269(IMAPve_g_Lrg_C1_BACK) -> IMAPve_g_Lrg_C1_BACK/1
  IMAP_Module/268(IMAPve_g_Lrg_C0_BACK) -> IMAPve_g_Lrg_C0_BACK/1
  SDFAve_g_Rrg_C3_BACK_COEF/1 -> IMAP_Module/182(SDFAve_g_Rrg_C3_BACK_COEF)
  SDFAve_g_Rrg_C0_BACK_COEF/1 -> IMAP_Module/179(SDFAve_g_Rrg_C0_BACK_COEF)
  SDFAve_g_Rrg_C1_BACK_COEF/1 -> IMAP_Module/180(SDFAve_g_Rrg_C1_BACK_COEF)
  SDFAve_y_Rrg_LINE_TYPE/1 -> IMAP_Module/186(SDFAve_y_Rrg_LINE_TYPE)
  SDFAve_g_Rrg_C2_BACK_COEF/1 -> IMAP_Module/181(SDFAve_g_Rrg_C2_BACK_COEF)
  SDFAve_g_Rrg_VIEW_RANGE_start/1 -> IMAP_Module/183(SDFAve_g_Rrg_VIEW_RANGE_start)
  SDFAve_g_Rrg_VIEW_RANGE_end/1 -> IMAP_Module/184(SDFAve_g_Rrg_VIEW_RANGE_end)
  SDFAve_y_Rrg_DETECT_QUALITY/1 -> IMAP_Module/185(SDFAve_y_Rrg_DETECT_QUALITY)
  SDFAve_y_Lrg_DETECT_QUALITY/1 -> IMAP_Module/177(SDFAve_y_Lrg_DETECT_QUALITY)
  SDFAve_g_Lrg_VIEW_RANGE_end/1 -> IMAP_Module/176(SDFAve_g_Lrg_VIEW_RANGE_end)
  SDFAve_g_Lrg_C1_BACK_COEF/1 -> IMAP_Module/172(SDFAve_g_Lrg_C1_BACK_COEF)
  SDFAve_g_Lrg_C3_BACK_COEF/1 -> IMAP_Module/174(SDFAve_g_Lrg_C3_BACK_COEF)
  SDFAve_g_Lrg_C2_BACK_COEF/1 -> IMAP_Module/173(SDFAve_g_Lrg_C2_BACK_COEF)
  SDFAve_g_Lrg_VIEW_RANGE_start/1 -> IMAP_Module/175(SDFAve_g_Lrg_VIEW_RANGE_start)
  SDFAve_g_Lrg_C0_BACK_COEF/1 -> IMAP_Module/171(SDFAve_g_Lrg_C0_BACK_COEF)
  SDFAve_y_Lrg_LINE_TYPE/1 -> IMAP_Module/178(SDFAve_y_Lrg_LINE_TYPE)
  IMAP_Module/54(IMAPve_d_BCM_HazardLamp_Switch) -> IMAPve_d_BCM_HazardLamp_Switch/1
  IMAP_Module/111(IMAPve_d_EMS_Gearbox_CtlAvail) -> IMAPve_d_EMS_Gearbox_CtlAvail/1
  IMAP_Module/142(IMAPve_d_TBOX_LocalTimeD) -> IMAPve_d_TBOX_LocalTimeD/1
  SDFAve_g_L0_C1_BACK_COEF/1 -> IMAP_Module/152(SDFAve_g_L0_C1_BACK_COEF)
  IMAP_Module/136(IMAPve_g_EPS_PowerCon) -> IMAPve_g_EPS_PowerCon/1
  IMAP_Module/130(IMAPve_d_EPB_Switch_State) -> IMAPve_d_EPB_Switch_State/1
  IMAP_Module/128(IMAPve_d_EPB_Display_Req) -> IMAPve_d_EPB_Display_Req/1
  IMAP_Module/69(IMAPve_d_EMS_AccPedal_Fault) -> IMAPve_d_EMS_AccPedal_Fault/1
  IMAP_Module/107(IMAPve_d_TCU_DCT_Clutch_State) -> IMAPve_d_TCU_DCT_Clutch_State/1
  IMAP_Module/105(IMAPve_d_TCU_AT_Failure) -> IMAPve_d_TCU_AT_Failure/1
  IMAP_Module/129(IMAPve_d_EPB_Warn_Req) -> IMAPve_d_EPB_Warn_Req/1
  IMAP_Module/21(IMAPve_d_EPS_LKA_State) -> IMAPve_d_EPS_LKA_State/1
  IMAP_Module/98(IMAPve_d_ESC_RL_WhlSpd_Fault) -> IMAPve_d_ESC_RL_WhlSpd_Fault/1
  IMAP_Module/96(IMAPve_d_ESC_FR_WhlSpd_Fault) -> IMAPve_d_ESC_FR_WhlSpd_Fault/1
  IMAP_Module/95(IMAPve_g_ESC_FR_WhlSpd) -> IMAPve_g_ESC_FR_WhlSpd/1
  IMAP_Module/94(IMAPve_d_ESC_FL_WhlSpd_Fault) -> IMAPve_d_ESC_FL_WhlSpd_Fault/1
  SDFAve_g_R0_C3_COEF/1 -> IMAP_Module/130(SDFAve_g_R0_C3_COEF)
  IMAP_Module/86(IMAPve_d_ESC_ABS_Active) -> IMAPve_d_ESC_ABS_Active/1
  IMAP_Module/83(IMAPve_d_ESC_MSR_Active) -> IMAPve_d_ESC_MSR_Active/1
  IMAP_Module/43(IMAPve_d_BCM_Left_Light) -> IMAPve_d_BCM_Left_Light/1
  SWINve_y_GW_Mp5_ISA_Switch/1 -> IMAP_Module/35(SWINve_y_GW_Mp5_ISA_Switch)
  IMAP_Module/80(IMAPve_d_ESC_OFF) -> IMAPve_d_ESC_OFF/1
  IMAP_Module/81(IMAPve_d_ESC_AlarmSig) -> IMAPve_d_ESC_AlarmSig/1
  IMAP_Module/133(IMAPve_d_ESC_Hold_State) -> IMAPve_d_ESC_Hold_State/1
  SWINve_y_Vehicle_detected_as_stationary/1 -> IMAP_Module/83(SWINve_y_Vehicle_detected_as_stationary)
  IMAP_Module/70(IMAPve_g_EMS_Driver_Torque) -> IMAPve_g_EMS_Driver_Torque/1
  IMAP_Module/169(IMAPve_g_ORI_L1_C1) -> IMAPve_g_ORI_L1_C1/1
  IMAP_Module/214(IMAPva_d_obj_MotionStatus) -> IMAPva_d_obj_MotionStatus/1
  IMAP_Module/213(IMAPva_d_obj_BrakeLight) -> IMAPva_d_obj_BrakeLight/1
  IMAP_Module/109(IMAPve_d_TCU_Select_ATMode) -> IMAPve_d_TCU_Select_ATMode/1
  IMAP_Module/207(IMAPva_g_obj_length) -> IMAPva_g_obj_length/1
  IMAP_Module/210(IMAPva_d_obj_status) -> IMAPva_d_obj_status/1
  IMAP_Module/153(IMAPva_d_ORI_Obj_Class) -> IMAPva_d_ORI_Obj_Class/1
  IMAP_Module/112(IMAPve_d_ESC_Brake_Failsafe) -> IMAPve_d_ESC_Brake_Failsafe/1
  IMAP_Module/149(IMAPve_g_GW_IC_Odometer) -> IMAPve_g_GW_IC_Odometer/1
  IMAP_Module/140(IMAPve_d_TBOX_LocalTimeY) -> IMAPve_d_TBOX_LocalTimeY/1
  IMAP_Module/197(IMAPva_g_obj_pos_x) -> IMAPva_g_obj_pos_x/1
  IMAP_Module/216(IMAPve_g_L0_C0) -> IMAPve_g_L0_C0/1
  IMAP_Module/101(IMAPve_d_ESC_FL_Wheel_Pulse) -> IMAPve_d_ESC_FL_Wheel_Pulse/1
  IMAP_Module/228(IMAPve_g_R0_VR) -> IMAPve_g_R0_VR/1
  SDFAve_g_L0_C2_BACK_COEF/1 -> IMAP_Module/153(SDFAve_g_L0_C2_BACK_COEF)
  IMAP_Module/202(IMAPva_g_obj_acc_y) -> IMAPva_g_obj_acc_y/1
  SWINve_y_Internal_SWS_status/1 -> IMAP_Module/47(SWINve_y_Internal_SWS_status)
  IMAP_Module/292(IMAPve_d_Camera_Status) -> IMAPve_d_Camera_Status/1
  IMAP_Module/125(IMAPve_d_BCM_LowBeam_State) -> IMAPve_d_BCM_LowBeam_State/1
  IMAP_Module/265(IMAPve_g_R1_C2_Back) -> IMAPve_g_R1_C2_Back/1
  IMAP_Module/92(IMAPve_d_ESC_RR_WheelPulVal) -> IMAPve_d_ESC_RR_WheelPulVal/1
  IMAP_Module/288(IMAPve_d_TSR_Sign_Type) -> IMAPve_d_TSR_Sign_Type/1
  IMAP_Module/73(IMAPve_d_ESC_Veh_Standstill) -> IMAPve_d_ESC_Veh_Standstill/1
  IMAP_Module/123(IMAPve_d_EMS_ACC_Inhibited) -> IMAPve_d_EMS_ACC_Inhibited/1
  IMAP_Module/160(IMAPve_g_ORI_L0_C3) -> IMAPve_g_ORI_L0_C3/1
  IMAP_Module/233(IMAPve_g_L1_C1) -> IMAPve_g_L1_C1/1
  IMAP_Module/284(IMAPve_d_Sign_ISA_Value) -> IMAPve_d_Sign_ISA_Value/1
  IMAP_Module/48(IMAPve_d_BCM_LF_Door_State) -> IMAPve_d_BCM_LF_Door_State/1
  IMAP_Module/184(IMAPve_g_ORI_R1_C0) -> IMAPve_g_ORI_R1_C0/1
  IMAP_Module/242(IMAPve_g_R1_C2) -> IMAPve_g_R1_C2/1
  SWINve_y_Rear_Left_pulse_malfunction/1 -> IMAP_Module/64(SWINve_y_Rear_Left_pulse_malfunction)
  IMAP_Module/217(IMAPve_g_L0_C1) -> IMAPve_g_L0_C1/1
  IMAP_Module/251(IMAPve_g_L0_C3_Back) -> IMAPve_g_L0_C3_Back/1
  IMAP_Module/226(IMAPve_g_R0_C2) -> IMAPve_g_R0_C2/1
  SDFAve_g_R1_C2_COEF/1 -> IMAP_Module/145(SDFAve_g_R1_C2_COEF)
  IMAP_Module/141(IMAPve_d_TBOX_LocalTimeM) -> IMAPve_d_TBOX_LocalTimeM/1
  IMAP_Module/263(IMAPve_g_R1_C0_Back) -> IMAPve_g_R1_C0_Back/1
  IMAP_Module/264(IMAPve_g_R1_C1_Back) -> IMAPve_g_R1_C1_Back/1
  IMAP_Module/91(IMAPve_d_ESC_RL_WheelPulVal) -> IMAPve_d_ESC_RL_WheelPulVal/1
  IMAP_Module/68(IMAPve_g_EMS_ACC_VirtualPedal) -> IMAPve_g_EMS_ACC_VirtualPedal/1
  IMAP_Module/116(IMAPve_d_ESC_ACC_Active) -> IMAPve_d_ESC_ACC_Active/1
  SDFAve_g_L1_MARK_WIDTH/1 -> IMAP_Module/142(SDFAve_g_L1_MARK_WIDTH)
  IMAP_Module/259(IMAPve_g_L1_C1_Back) -> IMAPve_g_L1_C1_Back/1
  IMAP_Module/267(IMAPve_g_R1_Range_Back) -> IMAPve_g_R1_Range_Back/1
  IMAP_Module/204(IMAPva_g_obj_pos_var_y) -> IMAPva_g_obj_pos_var_y/1
  IMAP_Module/260(IMAPve_g_L1_C2_Back) -> IMAPve_g_L1_C2_Back/1
  IMAP_Module/261(IMAPve_g_L1_C3_Back) -> IMAPve_g_L1_C3_Back/1
  IMAP_Module/77(IMAPve_d_BCM_Ignition_State) -> IMAPve_d_BCM_Ignition_State/1
  SWINve_y_ESP_in_regulation/1 -> IMAP_Module/27(SWINve_y_ESP_in_regulation)
  IMAP_Module/127(IMAPve_d_EPB_Status) -> IMAPve_d_EPB_Status/1
  SWINve_g_No_filtered_rear_left_speed/1 -> IMAP_Module/56(SWINve_g_No_filtered_rear_left_speed)
  IMAP_Module/258(IMAPve_g_L1_C0_Back) -> IMAPve_g_L1_C0_Back/1
  IMAP_Module/244(IMAPve_g_R1_VR) -> IMAPve_g_R1_VR/1
  IMAP_Module/134(IMAPve_d_EPS_Steer_Hold_State) -> IMAPve_d_EPS_Steer_Hold_State/1
  SWINve_y_State_indicating_steer_or_not/1 -> IMAP_Module/67(SWINve_y_State_indicating_steer_or_not)
  IMAP_Module/132(IMAPve_d_ESC_Drive_Direction) -> IMAPve_d_ESC_Drive_Direction/1
  IMAP_Module/143(IMAPve_d_TBOX_LocalTimeH) -> IMAPve_d_TBOX_LocalTimeH/1
  IMAP_Module/84(IMAPve_d_ESC_TCS_Active) -> IMAPve_d_ESC_TCS_Active/1
  IMAP_Module/18(IMAPve_d_DOW_Switch) -> IMAPve_d_DOW_Switch/1
  IMAP_Module/58(IMAPve_g_EMS_Pot_WhlT_Max) -> IMAPve_g_EMS_Pot_WhlT_Max/1
  IMAP_Module/252(IMAPve_g_L0_Range_Back) -> IMAPve_g_L0_Range_Back/1
  IMAP_Module/249(IMAPve_g_L0_C1_Back) -> IMAPve_g_L0_C1_Back/1
  IMAP_Module/199(IMAPva_g_obj_vel_x) -> IMAPva_g_obj_vel_x/1
  SWINve_g_Lateral_acceleration/1 -> IMAP_Module/48(SWINve_g_Lateral_acceleration)
  IMAP_Module/205(IMAPva_g_obj_pos_var_xy) -> IMAPva_g_obj_pos_var_xy/1
  IMAP_Module/243(IMAPve_g_R1_C3) -> IMAPve_g_R1_C3/1
  IMAP_Module/190(IMAPve_d_RF_Radar_Status) -> IMAPve_d_RF_Radar_Status/1
  IMAP_Module/246(IMAPve_d_R1_Type) -> IMAPve_d_R1_Type/1
  IMAP_Module/247(IMAPve_g_R1_W) -> IMAPve_g_R1_W/1
  IMAP_Module/241(IMAPve_g_R1_C1) -> IMAPve_g_R1_C1/1
  IMAP_Module/74(IMAPve_d_TCU_Actual_Gear) -> IMAPve_d_TCU_Actual_Gear/1
  IMAP_Module/206(IMAPva_g_obj_width) -> IMAPva_g_obj_width/1
  IMAP_Module/110(IMAPve_d_EMS_Engine_Status) -> IMAPve_d_EMS_Engine_Status/1
  IMAP_Module/238(IMAPve_d_L1_Type) -> IMAPve_d_L1_Type/1
  IMAP_Module/145(IMAPve_d_TBOX_LocalTimeS) -> IMAPve_d_TBOX_LocalTimeS/1
  IMAP_Module/13(IMAPve_d_ELK_Switch) -> IMAPve_d_ELK_Switch/1
  IMAP_Module/60(IMAPve_g_EMS_RealPedal) -> IMAPve_g_EMS_RealPedal/1
  IMAP_Module/97(IMAPve_g_ESC_RL_WhlSpd) -> IMAPve_g_ESC_RL_WhlSpd/1
  IMAP_Module/208(IMAPva_d_obj_class) -> IMAPva_d_obj_class/1
  IMAP_Module/11(IMAPve_d_ALC_TLC_Mode) -> IMAPve_d_ALC_TLC_Mode/1
  IMAP_Module/119(IMAPve_d_BCM_CHMSL_Status) -> IMAPve_d_BCM_CHMSL_Status/1
  SDFAve_g_L1_C0_BACK_COEF/1 -> IMAP_Module/161(SDFAve_g_L1_C0_BACK_COEF)
  IMAP_Module/157(IMAPva_g_ORI_Obj_RAngle) -> IMAPva_g_ORI_Obj_RAngle/1
  IMAP_Module/221(IMAPve_d_L0_Q) -> IMAPve_d_L0_Q/1
  IMAP_Module/19(IMAPve_d_JA_Brake_Switch) -> IMAPve_d_JA_Brake_Switch/1
  IMAP_Module/220(IMAPve_g_L0_VR) -> IMAPve_g_L0_VR/1
  SWINve_y_IC_FCW_Sensitivity/1 -> IMAP_Module/44(SWINve_y_IC_FCW_Sensitivity)
  IMAP_Module/158(IMAPva_g_ORI_Obj_Width) -> IMAPva_g_ORI_Obj_Width/1
  SWINve_g_EMS_Acceleration_pedal_position/1 -> IMAP_Module/15(SWINve_g_EMS_Acceleration_pedal_position)
  IMAP_Module/117(IMAPve_d_EMS_ACC_Effective) -> IMAPve_d_EMS_ACC_Effective/1
  IMAP_Module/170(IMAPve_g_ORI_L1_C0) -> IMAPve_g_ORI_L1_C0/1
  SDFAva_y_obj_BrakeLight/1 -> IMAP_Module/116(SDFAva_y_obj_BrakeLight)
  IMAP_Module/4(IMAPve_d_FCW_Switch) -> IMAPve_d_FCW_Switch/1
  IMAP_Module/168(IMAPve_g_ORI_L1_C2) -> IMAPve_g_ORI_L1_C2/1
  IMAP_Module/167(IMAPve_g_ORI_L1_C3) -> IMAPve_g_ORI_L1_C3/1
  IMAP_Module/151(IMAPve_d_ORI_CIPV_ID) -> IMAPve_d_ORI_CIPV_ID/1
  SDFAva_y_obj_lane/1 -> IMAP_Module/112(SDFAva_y_obj_lane)
  IMAP_Module/113(IMAPve_d_ESC_AEB_Available) -> IMAPve_d_ESC_AEB_Available/1
  IMAP_Module/147(IMAPve_d_Radar_State) -> IMAPve_d_Radar_State/1
  IMAP_Module/163(IMAPve_g_ORI_L0_C0) -> IMAPve_g_ORI_L0_C0/1
  IMAP_Module/215(IMAPve_d_Road_Type) -> IMAPve_d_Road_Type/1
  IMAP_Module/115(IMAPve_d_ESC_ACC_Available) -> IMAPve_d_ESC_ACC_Available/1
  IMAP_Module/124(IMAPve_d_EMS_Brake_Pedal) -> IMAPve_d_EMS_Brake_Pedal/1
  IMAP_Module/172(IMAPve_g_ORI_L1_VR) -> IMAPve_g_ORI_L1_VR/1
  IMAP_Module/256(IMAPve_g_R0_C3_Back) -> IMAPve_g_R0_C3_Back/1
  IMAP_Module/232(IMAPve_g_L1_C0) -> IMAPve_g_L1_C0/1
  IMAP_Module/156(IMAPva_g_ORI_Obj_LAngle) -> IMAPva_g_ORI_Obj_LAngle/1
  IMAP_Module/118(IMAPve_d_BCM_FrontWiper_State) -> IMAPve_d_BCM_FrontWiper_State/1
  IMAP_Module/155(IMAPva_g_ORI_Obj_LongDis) -> IMAPva_g_ORI_Obj_LongDis/1
  IMAP_Module/114(IMAPve_d_ESC_AEB_Active) -> IMAPve_d_ESC_AEB_Active/1
  IMAP_Module/154(IMAPva_g_ORI_Obj_RelVel) -> IMAPva_g_ORI_Obj_RelVel/1
  SDFAva_g_obj_vel_y/1 -> IMAP_Module/103(SDFAva_g_obj_vel_y)
  IMAP_Module/161(IMAPve_g_ORI_L0_C2) -> IMAPve_g_ORI_L0_C2/1
  IMAP_Module/150(IMAPve_d_Outside_Temp) -> IMAPve_d_Outside_Temp/1
  IMAP_Module/22(IMAPve_g_EPS_SW_Trq) -> IMAPve_g_EPS_SW_Trq/1
  IMAP_Module/229(IMAPve_d_R0_Q) -> IMAPve_d_R0_Q/1
  IMAP_Module/186(IMAPve_g_ORI_R1_VR) -> IMAPve_g_ORI_R1_VR/1
  IMAP_Module/257(IMAPve_g_R0_Range_Back) -> IMAPve_g_R0_Range_Back/1
  IMAP_Module/183(IMAPve_g_ORI_R1_C1) -> IMAPve_g_ORI_R1_C1/1
  IMAP_Module/182(IMAPve_g_ORI_R1_C2) -> IMAPve_g_ORI_R1_C2/1
  IMAP_Module/255(IMAPve_g_R0_C2_Back) -> IMAPve_g_R0_C2_Back/1
  IMAP_Module/181(IMAPve_g_ORI_R1_C3) -> IMAPve_g_ORI_R1_C3/1
  IMAP_Module/180(IMAPve_g_ORI_R0_W) -> IMAPve_g_ORI_R0_W/1
  SWINve_y_BCM_CHMSLStatus/1 -> IMAP_Module/6(SWINve_y_BCM_CHMSLStatus)
  SDFAva_g_obj_acc_x/1 -> IMAP_Module/104(SDFAva_g_obj_acc_x)
  SDFAve_y_ISAValue/1 -> IMAP_Module/187(SDFAve_y_ISAValue)
  IMAP_Module/178(IMAPve_d_ORI_R0_LT) -> IMAPve_d_ORI_R0_LT/1
  IMAP_Module/237(IMAPve_d_L1_Q) -> IMAPve_d_L1_Q/1
  IMAP_Module/159(IMAPva_d_ORI_Obj_ID) -> IMAPva_d_ORI_Obj_ID/1
  SDFAve_d_fusion_time_stamp/1 -> IMAP_Module/97(SDFAve_d_fusion_time_stamp)
  IMAP_Module/176(IMAPve_g_ORI_R0_C1) -> IMAPve_g_ORI_R0_C1/1
  IMAP_Module/40(IMAPve_g_SW_Angle) -> IMAPve_g_SW_Angle/1
  SDFAva_g_obj_length/1 -> IMAP_Module/110(SDFAva_g_obj_length)
  IMAP_Module/164(IMAPve_d_ORI_L0_Type) -> IMAPve_d_ORI_L0_Type/1
  IMAP_Module/148(IMAPve_d_Time_System_Clock) -> IMAPve_d_Time_System_Clock/1
  IMAP_Module/49(IMAPve_d_BCM_RF_Door_State) -> IMAPve_d_BCM_RF_Door_State/1
  IMAP_Module/195(IMAPve_d_obj_Num) -> IMAPve_d_obj_Num/1
  IMAP_Module/135(IMAPve_d_EPS_Warning_State) -> IMAPve_d_EPS_Warning_State/1
  IMAP_Module/194(IMAPve_d_Fusion_Time_Stamp) -> IMAPve_d_Fusion_Time_Stamp/1
  SDFAva_y_obj_class/1 -> IMAP_Module/111(SDFAva_y_obj_class)
  SDFAve_g_R1_C0_COEF/1 -> IMAP_Module/143(SDFAve_g_R1_C0_COEF)
  IMAP_Module/59(IMAPve_g_EMS_Pot_WhlT_Min) -> IMAPve_g_EMS_Pot_WhlT_Min/1
  IMAP_Module/191(IMAPve_d_LR_Radar_Status) -> IMAPve_d_LR_Radar_Status/1
  IMAP_Module/189(IMAPve_d_LF_Radar_Status) -> IMAPve_d_LF_Radar_Status/1
  IMAP_Module/137(IMAPve_d_ESC_EBD_AlarmSig) -> IMAPve_d_ESC_EBD_AlarmSig/1
  IMAP_Module/53(IMAPve_d_SCC_Right_SwitchSig) -> IMAPve_d_SCC_Right_SwitchSig/1
  SDFAve_y_L0_DETECT_QUALITY/1 -> IMAP_Module/124(SDFAve_y_L0_DETECT_QUALITY)
  IMAP_Module/55(IMAPve_d_PEPS_Door_Lock_Req) -> IMAPve_d_PEPS_Door_Lock_Req/1
  IMAP_Module/52(IMAPve_d_SCC_Left_SwitchSig) -> IMAPve_d_SCC_Left_SwitchSig/1
  SDFAve_y_R1_DETECT_QUALITY/1 -> IMAP_Module/148(SDFAve_y_R1_DETECT_QUALITY)
  SWINve_g_Steering_wheel_rotation_speed/1 -> IMAP_Module/71(SWINve_g_Steering_wheel_rotation_speed)
  IMAP_Module/103(IMAPve_d_ESC_RL_Wheel_Pulse) -> IMAPve_d_ESC_RL_Wheel_Pulse/1
  IMAP_Module/51(IMAPve_d_BCM_LR_Door_State) -> IMAPve_d_BCM_LR_Door_State/1
  SWINve_y_TCU_DCTClutchStatus/1 -> IMAP_Module/77(SWINve_y_TCU_DCTClutchStatus)
  SWINve_y_GW_SCC_LeftSteeringWheelSwitch/1 -> IMAP_Module/37(SWINve_y_GW_SCC_LeftSteeringWheelSwitch)
  IMAP_Module/29(IMAPve_d_ESC_LatAcc_Valid) -> IMAPve_d_ESC_LatAcc_Valid/1
  IMAP_Module/12(IMAPve_d_ESA_Switch) -> IMAPve_d_ESA_Switch/1
  IMAP_Module/162(IMAPve_g_ORI_L0_C1) -> IMAPve_g_ORI_L0_C1/1
  IMAP_Module/47(IMAPve_d_BCM_Trunk_State) -> IMAPve_d_BCM_Trunk_State/1
  IMAP_Module/235(IMAPve_g_L1_C3) -> IMAPve_g_L1_C3/1
  IMAP_Module/33(IMAPve_g_ESC_VehSpd) -> IMAPve_g_ESC_VehSpd/1
  IMAP_Module/90(IMAPve_d_ESC_FR_WheelPulVal) -> IMAPve_d_ESC_FR_WheelPulVal/1
  SWINve_y_TCU_PROGRAMME_ACC/1 -> IMAP_Module/80(SWINve_y_TCU_PROGRAMME_ACC)
  IMAP_Module/36(IMAPve_g_ESC_Brake_Press) -> IMAPve_g_ESC_Brake_Press/1
  SWINve_g_EMS_Driver_wheel_torque/1 -> IMAP_Module/19(SWINve_g_EMS_Driver_wheel_torque)
  IMAP_Module/179(IMAPve_g_ORI_R0_VR) -> IMAPve_g_ORI_R0_VR/1
  IMAP_Module/30(IMAPve_g_ESC_YawRate) -> IMAPve_g_ESC_YawRate/1
  IMAP_Module/42(IMAPve_d_BCM_HazardLamp) -> IMAPve_d_BCM_HazardLamp/1
  IMAP_Module/106(IMAPve_d_TCU_Shift_Valid) -> IMAPve_d_TCU_Shift_Valid/1
  IMAP_Module/122(IMAPve_d_EMS_ACC_CtlAvail) -> IMAPve_d_EMS_ACC_CtlAvail/1
  SDFAve_y_R0_DETECT_QUALITY/1 -> IMAP_Module/132(SDFAve_y_R0_DETECT_QUALITY)
  IMAP_Module/38(IMAPve_g_ESC_DySlope_Accuracy) -> IMAPve_g_ESC_DySlope_Accuracy/1
  IMAP_Module/31(IMAPve_d_ESC_YawRate_Valid) -> IMAPve_d_ESC_YawRate_Valid/1
  IMAP_Module/34(IMAPve_g_ESC_LonAcc) -> IMAPve_g_ESC_LonAcc/1
  IMAP_Module/28(IMAPve_g_ESC_LatAcc) -> IMAPve_g_ESC_LatAcc/1
  IMAP_Module/25(IMAPve_d_SAS_Trim_State) -> IMAPve_d_SAS_Trim_State/1
  IMAP_Module/185(IMAPve_d_ORI_R1_LT) -> IMAPve_d_ORI_R1_LT/1
  IMAP_Module/3(IMAPve_d_AEB_Switch) -> IMAPve_d_AEB_Switch/1
  SWINve_g_EMS_Driver_request/1 -> IMAP_Module/18(SWINve_g_EMS_Driver_request)
  SWINve_g_Vehicle_speed_of_wheelsensor/1 -> IMAP_Module/86(SWINve_g_Vehicle_speed_of_wheelsensor)
  IMAP_Module/27(IMAPve_g_EPS_LKA_Current) -> IMAPve_g_EPS_LKA_Current/1
  SDFAve_g_L0_C0_BACK_COEF/1 -> IMAP_Module/151(SDFAve_g_L0_C0_BACK_COEF)
  IMAP_Module/1(IMAPve_d_LKA_Main_Switch) -> IMAPve_d_LKA_Main_Switch/1
  SWINve_g_EMS_WhlTrq_max/1 -> IMAP_Module/23(SWINve_g_EMS_WhlTrq_max)
  IMAP_Module/15(IMAPve_d_BSD_LCW_Switch) -> IMAPve_d_BSD_LCW_Switch/1
  SWINve_y_State_of_EPS_for_LKA_function/1 -> IMAP_Module/68(SWINve_y_State_of_EPS_for_LKA_function)
  IMAP_Module/10(IMAPve_d_Speed_Limit) -> IMAPve_d_Speed_Limit/1
  IMAP_Module/5(IMAPve_d_FCW_Sensitivity) -> IMAPve_d_FCW_Sensitivity/1
  IMAP_Module/14(IMAPve_d_PEPS_RKE_Command) -> IMAPve_d_PEPS_RKE_Command/1
  IMAP_Module/166(IMAPve_g_ORI_L0_W) -> IMAPve_g_ORI_L0_W/1
  SDFAva_g_obj_width/1 -> IMAP_Module/109(SDFAva_g_obj_width)
  IMAP_Module/8(IMAPve_d_ISA_ISLC_Mode) -> IMAPve_d_ISA_ISLC_Mode/1
  IMAP_Module/102(IMAPve_d_ESC_FR_Wheel_Pulse) -> IMAPve_d_ESC_FR_Wheel_Pulse/1
  SDFAve_y_TSR_Sign_Type/1 -> IMAP_Module/191(SDFAve_y_TSR_Sign_Type)
  SWINve_y_EMS_ACCcontrol_Available/1 -> IMAP_Module/14(SWINve_y_EMS_ACCcontrol_Available)
  IMAP_Module/76(IMAPve_d_TCU_PRND_State) -> IMAPve_d_TCU_PRND_State/1
  SDFAve_d_R0_LINE_TYPE/1 -> IMAP_Module/133(SDFAve_d_R0_LINE_TYPE)
  SDFAve_g_R0_C3_BACK_COEF/1 -> IMAP_Module/159(SDFAve_g_R0_C3_BACK_COEF)
  SDFAve_g_CameraSignalFault/1 -> IMAP_Module/192(SDFAve_g_CameraSignalFault)
  IMAP_Module/201(IMAPva_g_obj_acc_x) -> IMAPva_g_obj_acc_x/1
  IMAP_Module/46(IMAPve_d_BCM_Opening_State) -> IMAPve_d_BCM_Opening_State/1
  IMAP_Module/165(IMAPve_g_ORI_L0_VR) -> IMAPve_g_ORI_L0_VR/1
  SDFAve_g_R1_C0_BACK_COEF/1 -> IMAP_Module/166(SDFAve_g_R1_C0_BACK_COEF)
  SDFAve_g_L0_BACK_RANGE/1 -> IMAP_Module/155(SDFAve_g_L0_BACK_RANGE)
  SDFAva_g_obj_pos_y/1 -> IMAP_Module/101(SDFAva_g_obj_pos_y)
  SDFAve_g_R0_C1_BACK_COEF/1 -> IMAP_Module/157(SDFAve_g_R0_C1_BACK_COEF)
  IMAP_Module/177(IMAPve_g_ORI_R0_C0) -> IMAPve_g_ORI_R0_C0/1
  IMAP_Module/240(IMAPve_g_R1_C0) -> IMAPve_g_R1_C0/1
  SDFAve_g_R0_C2_BACK_COEF/1 -> IMAP_Module/158(SDFAve_g_R0_C2_BACK_COEF)
  SDFAve_g_R1_MARK_WIDTH/1 -> IMAP_Module/150(SDFAve_g_R1_MARK_WIDTH)
  SWINve_y_GW_EMS_ACC_Ihibited_By_Engine/1 -> IMAP_Module/31(SWINve_y_GW_EMS_ACC_Ihibited_By_Engine)
  SWINve_y_Request_to_light_fault_lamp/1 -> IMAP_Module/66(SWINve_y_Request_to_light_fault_lamp)
  IMAP_Module/209(IMAPva_d_obj_lane) -> IMAPva_d_obj_lane/1
  SWINve_g_EMS_Actual_whlTrq/1 -> IMAP_Module/17(SWINve_g_EMS_Actual_whlTrq)
  SDFAve_g_L1_C1_BACK_COEF/1 -> IMAP_Module/162(SDFAve_g_L1_C1_BACK_COEF)
  IMAP_Module/32(IMAPve_g_ESC_UnYawRate) -> IMAPve_g_ESC_UnYawRate/1
  IMAP_Module/93(IMAPve_g_ESC_FL_WhlSpd) -> IMAPve_g_ESC_FL_WhlSpd/1
  IMAP_Module/192(IMAPve_d_RR_Radar_Status) -> IMAPve_d_RR_Radar_Status/1
  IMAP_Module/138(IMAPve_d_ESC_AVH_Status) -> IMAPve_d_ESC_AVH_Status/1
  SDFAve_g_L1_C2_BACK_COEF/1 -> IMAP_Module/163(SDFAve_g_L1_C2_BACK_COEF)
  IMAP_Module/87(IMAPve_d_ESC_ABS_Valid) -> IMAPve_d_ESC_ABS_Valid/1
  SDFAve_g_L1_BACK_RANGE/1 -> IMAP_Module/165(SDFAve_g_L1_BACK_RANGE)
  IMAP_Module/9(IMAPve_d_LDW_Warn_Mode) -> IMAPve_d_LDW_Warn_Mode/1
  SDFAve_g_R1_C3_COEF/1 -> IMAP_Module/146(SDFAve_g_R1_C3_COEF)
  SDFAve_g_L1_C2_COEF/1 -> IMAP_Module/137(SDFAve_g_L1_C2_COEF)
  SDFAve_g_R1_C2_BACK_COEF/1 -> IMAP_Module/168(SDFAve_g_R1_C2_BACK_COEF)
  IMAP_Module/234(IMAPve_g_L1_C2) -> IMAPve_g_L1_C2/1
  SDFAve_g_R1_VIEW_RANGE/1 -> IMAP_Module/147(SDFAve_g_R1_VIEW_RANGE)
  SDFAve_g_L1_C0_COEF/1 -> IMAP_Module/135(SDFAve_g_L1_C0_COEF)
  SDFAve_g_R1_C1_COEF/1 -> IMAP_Module/144(SDFAve_g_R1_C1_COEF)
  IMAP_Module/253(IMAPve_g_R0_C0_Back) -> IMAPve_g_R0_C0_Back/1
  IMAP_Module/174(IMAPve_g_ORI_R0_C3) -> IMAPve_g_ORI_R0_C3/1
  SDFAve_g_R0_C1_COEF/1 -> IMAP_Module/128(SDFAve_g_R0_C1_COEF)
  SDFAve_d_R1_LINE_TYPE/1 -> IMAP_Module/149(SDFAve_d_R1_LINE_TYPE)
  IMAP_Module/37(IMAPve_g_ESC_Static_Slope) -> IMAPve_g_ESC_Static_Slope/1
  SDFAve_d_L0_LINE_TYPE/1 -> IMAP_Module/125(SDFAve_d_L0_LINE_TYPE)
  IMAP_Module/2(IMAPve_d_LKA_Mode) -> IMAPve_d_LKA_Mode/1
  SDFAve_g_L1_C1_COEF/1 -> IMAP_Module/136(SDFAve_g_L1_C1_COEF)
  SWINve_g_GW_EMS_Pot_WhlTrq_Min/1 -> IMAP_Module/34(SWINve_g_GW_EMS_Pot_WhlTrq_Min)
  SDFAve_g_L0_C3_COEF/1 -> IMAP_Module/122(SDFAve_g_L0_C3_COEF)
  SDFAve_g_L0_C2_COEF/1 -> IMAP_Module/121(SDFAve_g_L0_C2_COEF)
  SDFAve_y_ROAD_TYPE/1 -> IMAP_Module/118(SDFAve_y_ROAD_TYPE)
  SDFAve_d_sen_sta_RB_radar/1 -> IMAP_Module/95(SDFAve_d_sen_sta_RB_radar)
  SDFAve_g_R0_C2_COEF/1 -> IMAP_Module/129(SDFAve_g_R0_C2_COEF)
  SDFAve_g_R0_BACK_RANGE/1 -> IMAP_Module/160(SDFAve_g_R0_BACK_RANGE)
  SDFAve_g_L0_MARK_WIDTH/1 -> IMAP_Module/126(SDFAve_g_L0_MARK_WIDTH)
  SDFAve_g_L0_C1_COEF/1 -> IMAP_Module/120(SDFAve_g_L0_C1_COEF)
  IMAP_Module/100(IMAPve_d_ESC_RR_WhlSpd_Fault) -> IMAPve_d_ESC_RR_WhlSpd_Fault/1
  SDFAve_g_R0_VIEW_RANGE/1 -> IMAP_Module/131(SDFAve_g_R0_VIEW_RANGE)
  SDFAve_g_L0_VIEW_RANGE/1 -> IMAP_Module/123(SDFAve_g_L0_VIEW_RANGE)
  IMAP_Module/196(IMAPva_d_obj_id) -> IMAPva_d_obj_id/1
  SDFAve_d_sensor_status/1 -> IMAP_Module/91(SDFAve_d_sensor_status)
  SWINve_g_No_filtered_front_right_speed/1 -> IMAP_Module/55(SWINve_g_No_filtered_front_right_speed)
  IMAP_Module/108(IMAPve_d_TCU_Gear_Engage) -> IMAPve_d_TCU_Gear_Engage/1
  SWINve_y_Dynamic_slope_accuracy/1 -> IMAP_Module/12(SWINve_y_Dynamic_slope_accuracy)
  SDFAva_d_obj_age/1 -> IMAP_Module/114(SDFAva_d_obj_age)
  SDFAve_g_L1_C3_BACK_COEF/1 -> IMAP_Module/164(SDFAve_g_L1_C3_BACK_COEF)
  SDFAva_d_obj_status/1 -> IMAP_Module/113(SDFAva_d_obj_status)
  SDFAva_g_obj_pos_x/1 -> IMAP_Module/100(SDFAva_g_obj_pos_x)
  SDFAva_g_obj_pos_var_y/1 -> IMAP_Module/107(SDFAva_g_obj_pos_var_y)
  IMAP_Module/139(IMAPve_g_BCM_Battery_Voltage) -> IMAPve_g_BCM_Battery_Voltage/1
  SDFAva_g_obj_vel_x/1 -> IMAP_Module/102(SDFAva_g_obj_vel_x)
  IMAP_Module/289(IMAPve_g_Camera_Signal_Fault) -> IMAPve_g_Camera_Signal_Fault/1
  SDFAve_g_R0_C0_BACK_COEF/1 -> IMAP_Module/156(SDFAve_g_R0_C0_BACK_COEF)
  IMAP_Module/6(IMAPve_d_ISA_Switch) -> IMAPve_d_ISA_Switch/1
  IMAP_Module/262(IMAPve_g_L1_Range_Back) -> IMAPve_g_L1_Range_Back/1
  SDFAva_y_obj_id/1 -> IMAP_Module/99(SDFAva_y_obj_id)
  SDFAve_d_obj_Num/1 -> IMAP_Module/98(SDFAve_d_obj_Num)
  IMAP_Module/218(IMAPve_g_L0_C2) -> IMAPve_g_L0_C2/1
  SWINve_g_No_filtered_rear_rignt_speed/1 -> IMAP_Module/57(SWINve_g_No_filtered_rear_rignt_speed)
  SDFAve_d_sen_sta_LF_radar/1 -> IMAP_Module/92(SDFAve_d_sen_sta_LF_radar)
  SDFAva_y_obj_MotionStatus/1 -> IMAP_Module/117(SDFAva_y_obj_MotionStatus)
  SDFAve_g_R1_C1_BACK_COEF/1 -> IMAP_Module/167(SDFAve_g_R1_C1_BACK_COEF)
  SDFAve_g_L1_VIEW_RANGE/1 -> IMAP_Module/139(SDFAve_g_L1_VIEW_RANGE)
  SDFAve_d_L1_LINE_TYPE/1 -> IMAP_Module/141(SDFAve_d_L1_LINE_TYPE)
  IMAP_Module/99(IMAPve_g_ESC_RR_WhlSpd) -> IMAPve_g_ESC_RR_WhlSpd/1
  IMAP_Module/222(IMAPve_d_L0_Type) -> IMAPve_d_L0_Type/1
  IMAP_Module/24(IMAPve_d_SAS_Clb_State) -> IMAPve_d_SAS_Clb_State/1
  SWINve_y_BCM_BrakeLampStatus/1 -> IMAP_Module/5(SWINve_y_BCM_BrakeLampStatus)
  IMAP_Module/188(IMAPve_d_Sensor_Status) -> IMAPve_d_Sensor_Status/1
  IMAP_Module/144(IMAPve_d_TBOX_LocalTimeMin) -> IMAPve_d_TBOX_LocalTimeMin/1
  IMAP_Module/224(IMAPve_g_R0_C0) -> IMAPve_g_R0_C0/1
  SWINve_y_SWS_calibration/1 -> IMAP_Module/73(SWINve_y_SWS_calibration)
  IMAP_Module/88(IMAPve_d_ESC_ABS_AlarmSig) -> IMAPve_d_ESC_ABS_AlarmSig/1
  SDFAve_g_L1_C3_COEF/1 -> IMAP_Module/138(SDFAve_g_L1_C3_COEF)
  IMAP_Module/152(IMAPve_d_ORI_Obj_Num) -> IMAPve_d_ORI_Obj_Num/1
  IMAP_Module/173(IMAPve_g_ORI_L1_W) -> IMAPve_g_ORI_L1_W/1
  IMAP_Module/35(IMAPve_d_ESC_LonAcc_Valid) -> IMAPve_d_ESC_LonAcc_Valid/1
  SDFAve_g_R1_C3_BACK_COEF/1 -> IMAP_Module/169(SDFAve_g_R1_C3_BACK_COEF)
  SWINve_g_YawRate_Raw/1 -> IMAP_Module/89(SWINve_g_YawRate_Raw)
  SWINve_y_Vehiclespd_unavailability_flag/1 -> IMAP_Module/87(SWINve_y_Vehiclespd_unavailability_flag)
  IMAP_Module/131(IMAPve_d_EPB_Switch_Valid) -> IMAPve_d_EPB_Switch_Valid/1
  IMAP_Module/245(IMAPve_d_R1_Q) -> IMAPve_d_R1_Q/1
  SDFAva_g_obj_pos_var_x/1 -> IMAP_Module/106(SDFAva_g_obj_pos_var_x)
  SWINve_y_IC_Fcw_Activation_Config/1 -> IMAP_Module/43(SWINve_y_IC_Fcw_Activation_Config)
  IMAP_Module/212(IMAPva_d_obj_TurnLight) -> IMAPva_d_obj_TurnLight/1
  IMAP_Module/236(IMAPve_g_L1_VR) -> IMAPve_g_L1_VR/1
  IMAP_Module/121(IMAPve_d_ACU_Passenger_Belt) -> IMAPve_d_ACU_Passenger_Belt/1
  System_Clock/1 -> IMAP_Module/90(System_Clock)
  IMAP_Module/126(IMAPve_d_BCM_HighBeam_State) -> IMAPve_d_BCM_HighBeam_State/1
  IMAP_Module/219(IMAPve_g_L0_C3) -> IMAPve_g_L0_C3/1
  IMAP_Module/248(IMAPve_g_L0_C0_Back) -> IMAPve_g_L0_C0_Back/1
  IMAP_Module/175(IMAPve_g_ORI_R0_C2) -> IMAPve_g_ORI_R0_C2/1
  SWINve_y_Vehicle_Hold_Status/1 -> IMAP_Module/85(SWINve_y_Vehicle_Hold_Status)
  SDFAve_g_R0_C0_COEF/1 -> IMAP_Module/127(SDFAve_g_R0_C0_COEF)
  SWINve_y_Torque_limitation_if_DAE_limit/1 -> IMAP_Module/82(SWINve_y_Torque_limitation_if_DAE_limit)
  SWINve_y_TCU_Gear_lever_position/1 -> IMAP_Module/78(SWINve_y_TCU_Gear_lever_position)
  SWINve_y_Vehicle_driving_direction/1 -> IMAP_Module/84(SWINve_y_Vehicle_driving_direction)
  SDFAva_g_obj_acc_y/1 -> IMAP_Module/105(SDFAva_g_obj_acc_y)
  IMAP_Module/41(IMAPve_g_SW_Angle_Speed) -> IMAPve_g_SW_Angle_Speed/1
  SWINve_y_Brake_secondary_contact/1 -> IMAP_Module/9(SWINve_y_Brake_secondary_contact)
  SWINve_y_LKA_main_switch/1 -> IMAP_Module/50(SWINve_y_LKA_main_switch)
  SWINve_y_TCU_AGB_Target_position/1 -> IMAP_Module/75(SWINve_y_TCU_AGB_Target_position)
  SWINve_g_TMC_pressure/1 -> IMAP_Module/81(SWINve_g_TMC_pressure)
  SWINve_g_Steering_wheel_angle/1 -> IMAP_Module/70(SWINve_g_Steering_wheel_angle)
  SWINve_y_TCU_GearEngagement/1 -> IMAP_Module/79(SWINve_y_TCU_GearEngagement)
  IMAP_Module/82(IMAPve_d_ESC_ESC_Active) -> IMAPve_d_ESC_ESC_Active/1
  SWINve_y_MSR_in_regulation/1 -> IMAP_Module/53(SWINve_y_MSR_in_regulation)
  SWINve_y_TCU_ATFailure/1 -> IMAP_Module/76(SWINve_y_TCU_ATFailure)
  SWINve_y_LC_Mode/1 -> IMAP_Module/49(SWINve_y_LC_Mode)
  SWINve_y_ABS_in_regulation/1 -> IMAP_Module/1(SWINve_y_ABS_in_regulation)
  IMAP_Module/227(IMAPve_g_R0_C3) -> IMAPve_g_R0_C3/1
  IMAP_Module/56(IMAPve_d_BCM_Door_Lock_State) -> IMAPve_d_BCM_Door_Lock_State/1
  SWINve_g_number_of_kilometer/1 -> IMAP_Module/58(SWINve_g_number_of_kilometer)
  IMAP_Module/171(IMAPve_d_ORI_L1_Type) -> IMAPve_d_ORI_L1_Type/1
  SWINve_y_Rear_Right_pulse_malfunction/1 -> IMAP_Module/65(SWINve_y_Rear_Right_pulse_malfunction)
  IMAP_Module/146(IMAPve_d_TBOX_LocalTime_Valid) -> IMAPve_d_TBOX_LocalTime_Valid/1
  SWINve_y_MP5_AEB_Activation_Config/1 -> IMAP_Module/52(SWINve_y_MP5_AEB_Activation_Config)
  IMAP_Module/120(IMAPve_d_BCM_BrakeLamp_State) -> IMAPve_d_BCM_BrakeLamp_State/1
  SWINve_g_Pulse_counter_front_right_wheel/1 -> IMAP_Module/61(SWINve_g_Pulse_counter_front_right_wheel)
  SWINve_g_Steering_wheel_torque/1 -> IMAP_Module/72(SWINve_g_Steering_wheel_torque)
  SWINve_y_Park_brake_function_status/1 -> IMAP_Module/59(SWINve_y_Park_brake_function_status)
  SWINve_g_No_filtered_front_left_speed/1 -> IMAP_Module/54(SWINve_g_No_filtered_front_left_speed)
  SWINve_g_Pulse_counter_rearleft_wheel/1 -> IMAP_Module/62(SWINve_g_Pulse_counter_rearleft_wheel)
  SWINve_g_Pulse_counter_front_left_wheel/1 -> IMAP_Module/60(SWINve_g_Pulse_counter_front_left_wheel)
  SWINve_y_GW_EMS_EMS_Status_ACC/1 -> IMAP_Module/32(SWINve_y_GW_EMS_EMS_Status_ACC)
  SWINve_y_IC_passengerBeltSwitchSig/1 -> IMAP_Module/45(SWINve_y_IC_passengerBeltSwitchSig)
  SWINve_y_High_beam_state/1 -> IMAP_Module/42(SWINve_y_High_beam_state)
  SWINve_y_GW_Mp5_TSR_Switch/1 -> IMAP_Module/36(SWINve_y_GW_Mp5_TSR_Switch)
  SWINve_y_IC_seat_bealt_driver_state/1 -> IMAP_Module/46(SWINve_y_IC_seat_bealt_driver_state)
  IMAP_Module/223(IMAPve_g_L0_W) -> IMAPve_g_L0_W/1
  IMAP_Module/39(IMAPve_g_ESC_DySlope) -> IMAPve_g_ESC_DySlope/1
  SWINve_g_EMS_WhlTrq_min/1 -> IMAP_Module/25(SWINve_g_EMS_WhlTrq_min)
  IMAP_Module/44(IMAPve_d_BCM_Right_Light) -> IMAPve_d_BCM_Right_Light/1
  SDFAve_g_R1_BACK_RANGE/1 -> IMAP_Module/170(SDFAve_g_R1_BACK_RANGE)
  IMAP_Module/104(IMAPve_d_ESC_RR_Wheel_Pulse) -> IMAPve_d_ESC_RR_Wheel_Pulse/1
  IMAP_Module/23(IMAPve_d_EPS_Trq_State) -> IMAPve_d_EPS_Trq_State/1
  SWINve_y_GW_SCC_RightSteeringWheelSwitch/1 -> IMAP_Module/38(SWINve_y_GW_SCC_RightSteeringWheelSwitch)
  IMAP_Module/266(IMAPve_g_R1_C3_Back) -> IMAPve_g_R1_C3_Back/1
  IMAP_Module/187(IMAPve_g_ORI_R1_W) -> IMAPve_g_ORI_R1_W/1
  SWINve_y_EMS_GearBox_ACC_Ctl_Available/1 -> IMAP_Module/22(SWINve_y_EMS_GearBox_ACC_Ctl_Available)
  SDFAva_g_obj_pos_var_xy/1 -> IMAP_Module/108(SDFAva_g_obj_pos_var_xy)
  SWINve_y_EMS_Engine_state/1 -> IMAP_Module/21(SWINve_y_EMS_Engine_state)
  SWINve_y_Braking_effort/1 -> IMAP_Module/10(SWINve_y_Braking_effort)
  IMAP_Module/239(IMAPve_g_L1_W) -> IMAPve_g_L1_W/1
  SWINve_y_GW_BCM_SEV_main_state/1 -> IMAP_Module/30(SWINve_y_GW_BCM_SEV_main_state)
  SWINve_y_Dynamic_slope/1 -> IMAP_Module/11(SWINve_y_Dynamic_slope)
  SWINve_g_EMS_WhlTrq_min_offset/1 -> IMAP_Module/26(SWINve_g_EMS_WhlTrq_min_offset)
  SWINve_y_ASR_in_regulation/1 -> IMAP_Module/4(SWINve_y_ASR_in_regulation)
  SWINve_y_ASR_ESP_disconnected/1 -> IMAP_Module/3(SWINve_y_ASR_ESP_disconnected)
  SWINve_g_GW_EMS_Pot_WhlTrq_Max/1 -> IMAP_Module/33(SWINve_g_GW_EMS_Pot_WhlTrq_Max)
  SWINve_g_Yaw_speed/1 -> IMAP_Module/88(SWINve_g_Yaw_speed)
  IMAP_Module/254(IMAPve_g_R0_C1_Back) -> IMAPve_g_R0_C1_Back/1
  SWINve_g_EMS_Engine_RPM/1 -> IMAP_Module/20(SWINve_g_EMS_Engine_RPM)
  SWINve_y_BCM_State_Front_Wiper/1 -> IMAP_Module/7(SWINve_y_BCM_State_Front_Wiper)
  SWINve_y_EMS_ACC_Effecitive_EMS/1 -> IMAP_Module/13(SWINve_y_EMS_ACC_Effecitive_EMS)
  SWINve_y_Message_from_ESC_informing/1 -> IMAP_Module/51(SWINve_y_Message_from_ESC_informing)
  SDFAve_g_R0_MARK_WIDTH/1 -> IMAP_Module/134(SDFAve_g_R0_MARK_WIDTH)
  IMAP_Module/17(IMAPve_d_RCTA_Swtich) -> IMAPve_d_RCTA_Swtich/1
  SWINve_g_ACCEL_LONGI_CALIB/1 -> IMAP_Module/2(SWINve_g_ACCEL_LONGI_CALIB)
  SWINve_y_BCM_Status_Indicator/1 -> IMAP_Module/8(SWINve_y_BCM_Status_Indicator)
  IMAP_Module/203(IMAPva_g_obj_pos_var_x) -> IMAPva_g_obj_pos_var_x/1
  IMAP_Module/16(IMAPve_d_FCTA_Switch) -> IMAPve_d_FCTA_Switch/1
  IMAP_Module/250(IMAPve_g_L0_C2_Back) -> IMAPve_g_L0_C2_Back/1
  SDFAve_d_sen_sta_LB_radar/1 -> IMAP_Module/94(SDFAve_d_sen_sta_LB_radar)
  SWINve_g_EMS_WhlTrq_max_offset/1 -> IMAP_Module/24(SWINve_g_EMS_WhlTrq_max_offset)
  IMAP_Module/85(IMAPve_d_ESC_VehSpd_Valid) -> IMAPve_d_ESC_VehSpd_Valid/1
  SWINve_g_Pulse_counter_rearright_wheel/1 -> IMAP_Module/63(SWINve_g_Pulse_counter_rearright_wheel)
  IMAP_Module/61(IMAPve_g_EMS_MaxTWhl) -> IMAPve_g_EMS_MaxTWhl/1
  IMAP_Module/72(IMAPve_g_EMS_Engine_Speed) -> IMAPve_g_EMS_Engine_Speed/1
  IMAP_Module/26(IMAPve_d_EPS_TrqLim_State) -> IMAPve_d_EPS_TrqLim_State/1
  SDFAve_y_L1_DETECT_QUALITY/1 -> IMAP_Module/140(SDFAve_y_L1_DETECT_QUALITY)
  IMAP_Module/71(IMAPve_d_ESC_Brake_Effort) -> IMAPve_d_ESC_Brake_Effort/1
  IMAP_Module/198(IMAPva_g_obj_pos_y) -> IMAPva_g_obj_pos_y/1
  IMAP_Module/7(IMAPve_d_TSR_Switch) -> IMAPve_d_TSR_Switch/1
  IMAP_Module/57(IMAPve_d_EMS_ACC_Status) -> IMAPve_d_EMS_ACC_Status/1
  SWINve_y_Front_right_pulse_malfunction/1 -> IMAP_Module/29(SWINve_y_Front_right_pulse_malfunction)
  IMAP_Module/67(IMAPve_g_EMS_Realize_TWhl) -> IMAPve_g_EMS_Realize_TWhl/1
  IMAP_Module/63(IMAPve_g_EMS_MinTWhl) -> IMAPve_g_EMS_MinTWhl/1
  IMAP_Module/79(IMAPve_d_SWS_Failure_Status) -> IMAPve_d_SWS_Failure_Status/1
  IMAP_Module/20(IMAPve_d_JA_Alert_Switch) -> IMAPve_d_JA_Alert_Switch/1
  SWINve_g_EMS_Actual_torque/1 -> IMAP_Module/16(SWINve_g_EMS_Actual_torque)
  IMAP_Module/89(IMAPve_d_ESC_FL_WheelPulVal) -> IMAPve_d_ESC_FL_WheelPulVal/1
  IMAP_Module/65(IMAPve_g_EMS_Actual_FlwT) -> IMAPve_g_EMS_Actual_FlwT/1
  IMAP_Module/211(IMAPva_d_obj_age) -> IMAPva_d_obj_age/1
  IMAP_Module/64(IMAPve_g_EMS_MinTWhl_Offset) -> IMAPve_g_EMS_MinTWhl_Offset/1
  IMAP_Module/200(IMAPva_g_obj_vel_y) -> IMAPva_g_obj_vel_y/1
  SWINve_g_Static_slope/1 -> IMAP_Module/69(SWINve_g_Static_slope)
  IMAP_Module/78(IMAPve_d_ACU_Driver_Belt) -> IMAPve_d_ACU_Driver_Belt/1
  SDFAve_g_L0_C0_COEF/1 -> IMAP_Module/119(SDFAve_g_L0_C0_COEF)
  SWINve_y_Front_Left_pulse_malfunction/1 -> IMAP_Module/28(SWINve_y_Front_Left_pulse_malfunction)
  SDFAva_y_obj_TurnLight/1 -> IMAP_Module/115(SDFAva_y_obj_TurnLight)
  IMAP_Module/225(IMAPve_g_R0_C1) -> IMAPve_g_R0_C1/1
  IMAP_Module/50(IMAPve_d_BCM_RR_Door_State) -> IMAPve_d_BCM_RR_Door_State/1
  IMAP_Module/75(IMAPve_d_TCU_Target_Gear) -> IMAPve_d_TCU_Target_Gear/1
  SWINve_y_SWS_trim/1 -> IMAP_Module/74(SWINve_y_SWS_trim)
  IMAP_Module/230(IMAPve_d_R0_Type) -> IMAPve_d_R0_Type/1
  SDFAve_g_L0_C3_BACK_COEF/1 -> IMAP_Module/154(SDFAve_g_L0_C3_BACK_COEF)
  IMAP_Module/231(IMAPve_g_R0_W) -> IMAPve_g_R0_W/1
  IMAP_Module/66(IMAPve_g_EMS_Actual_IndT) -> IMAPve_g_EMS_Actual_IndT/1
  IMAP_Module/45(IMAPve_d_ESC_BrakeLamp_Req) -> IMAPve_d_ESC_BrakeLamp_Req/1
  IMAP_Module/62(IMAPve_g_EMS_MaxTWhl_Offset) -> IMAPve_g_EMS_MaxTWhl_Offset/1
  SDFAve_d_sen_sta_RF_radar/1 -> IMAP_Module/93(SDFAve_d_sen_sta_RF_radar)
  SWINve_y_EPS_ESAState/1 -> IMAP_Module/206(SWINve_y_EPS_ESAState)
  SWINve_y_MP5_APAModeSelect/1 -> IMAP_Module/217(SWINve_y_MP5_APAModeSelect)
  SWINve_y_MP5_WorkSt/1 -> IMAP_Module/216(SWINve_y_MP5_WorkSt)
  SWINve_y_MP5_DMS_SmokingMonitor/1 -> IMAP_Module/230(SWINve_y_MP5_DMS_SmokingMonitor)
  SWINve_y_MP5_DMS_EyeFatigueMonitor/1 -> IMAP_Module/226(SWINve_y_MP5_DMS_EyeFatigueMonitor)
  SWINve_y_MP5_DMS_LongtimeDriveMonitor/1 -> IMAP_Module/227(SWINve_y_MP5_DMS_LongtimeDriveMonitor)
  SWINve_y_MP5_UPASwitch/1 -> IMAP_Module/219(SWINve_y_MP5_UPASwitch)
  SWINve_y_MP5_DMS_SystemEnable/1 -> IMAP_Module/223(SWINve_y_MP5_DMS_SystemEnable)
  SWINve_y_BCM_FrontWiperSwitchSt/1 -> IMAP_Module/214(SWINve_y_BCM_FrontWiperSwitchSt)
  SWINve_y_MP5_LanguageSet/1 -> IMAP_Module/218(SWINve_y_MP5_LanguageSet)
  SWINve_y_ESC_TCSErrorStatus/1 -> IMAP_Module/198(SWINve_y_ESC_TCSErrorStatus)
  SWINve_y_BCM_LeftTurnSwitchSt/1 -> IMAP_Module/212(SWINve_y_BCM_LeftTurnSwitchSt)
  SWINve_y_ESC_RRWDirection/1 -> IMAP_Module/200(SWINve_y_ESC_RRWDirection)
  SWINve_y_BCM_IHBC_Function_Enabled/1 -> IMAP_Module/215(SWINve_y_BCM_IHBC_Function_Enabled)
  SWINve_y_ACU_RearRightBeltSwitchSig/1 -> IMAP_Module/209(SWINve_y_ACU_RearRightBeltSwitchSig)
  SWINve_y_MP5_DMS_MessageType/1 -> IMAP_Module/222(SWINve_y_MP5_DMS_MessageType)
  SWINve_y_EPS_SteeringAngle_Flag/1 -> IMAP_Module/202(SWINve_y_EPS_SteeringAngle_Flag)
  SWINve_g_EPS_SteeringAngle/1 -> IMAP_Module/203(SWINve_g_EPS_SteeringAngle)
  SWINve_y_ACU_RearMiddleBeltSwitchSig/1 -> IMAP_Module/208(SWINve_y_ACU_RearMiddleBeltSwitchSig)
  SWINve_y_MP5_DMS_Sensity/1 -> IMAP_Module/225(SWINve_y_MP5_DMS_Sensity)
  SWINve_y_MP5_DMS_DeleteUserNum/1 -> IMAP_Module/224(SWINve_y_MP5_DMS_DeleteUserNum)
  SWINve_y_EPS_DriverOverride/1 -> IMAP_Module/204(SWINve_y_EPS_DriverOverride)
  SWINve_y_ESC_EPBErrorStatus/1 -> IMAP_Module/201(SWINve_y_ESC_EPBErrorStatus)
  SWINve_y_MP5_DMS_UsingPhoneMonitor/1 -> IMAP_Module/229(SWINve_y_MP5_DMS_UsingPhoneMonitor)
  SWINve_y_MP5_AutoPilotSwitch/1 -> IMAP_Module/221(SWINve_y_MP5_AutoPilotSwitch)
  SWINve_y_ESC_FRWDirection/1 -> IMAP_Module/197(SWINve_y_ESC_FRWDirection)
  SWINve_y_ESC_FLWDirection/1 -> IMAP_Module/196(SWINve_y_ESC_FLWDirection)
  SWINve_y_MP5_DMS_DrinkWaterMonitor/1 -> IMAP_Module/231(SWINve_y_MP5_DMS_DrinkWaterMonitor)
  SWINve_y_EMS_PowertrainControlSt/1 -> IMAP_Module/210(SWINve_y_EMS_PowertrainControlSt)
  SWINve_y_TCU_TCUAvailable/1 -> IMAP_Module/211(SWINve_y_TCU_TCUAvailable)
  SWINve_y_ESC-RLWDirection/1 -> IMAP_Module/199(SWINve_y_ESC-RLWDirection)
  SWINve_y_MP5_DMS_SideViewMonitor/1 -> IMAP_Module/228(SWINve_y_MP5_DMS_SideViewMonitor)
  SWINve_y_BCM_RightTurnSwitchSt/1 -> IMAP_Module/213(SWINve_y_BCM_RightTurnSwitchSt)
  SWINve_y_EPS_DriverInitializedESA/1 -> IMAP_Module/205(SWINve_y_EPS_DriverInitializedESA)
  SWINve_y_MP5_DMS_UserAccount/1 -> IMAP_Module/232(SWINve_y_MP5_DMS_UserAccount)
  SWINve_y_ACU_RearLeftBeltSwitchSig/1 -> IMAP_Module/207(SWINve_y_ACU_RearLeftBeltSwitchSig)
  SWINve_y_MP5_FLKActivation/1 -> IMAP_Module/220(SWINve_y_MP5_FLKActivation)
  IMAP_Module/307(IMAPve_d_EMS_PowertrainCtl_State) -> IMAPve_d_EMS_PowertrainCtl_State/1
  IMAP_Module/297(IMAPve_d_ESC_RRW_Direction) -> IMAPve_d_ESC_RRW_Direction/1
  IMAP_Module/299(IMAPve_d_EPS_SteeringAngle_Flag) -> IMAPve_d_EPS_SteeringAngle_Flag/1
  IMAP_Module/300(IMAPve_g_EPS_SteeringAngle) -> IMAPve_g_EPS_SteeringAngle/1
  IMAP_Module/316(IMAPve_d_MP5_UPA_Switch) -> IMAPve_d_MP5_UPA_Switch/1
  IMAP_Module/315(IMAPve_d_MP5_LanguageSet) -> IMAPve_d_MP5_LanguageSet/1
  IMAP_Module/314(IMAPve_d_MP5_APA_ModeSelect) -> IMAPve_d_MP5_APA_ModeSelect/1
  IMAP_Module/327(IMAPve_d_MP5_DMS_Smoking) -> IMAPve_d_MP5_DMS_Smoking/1
  IMAP_Module/325(IMAPve_d_MP5_DMS_SideView) -> IMAPve_d_MP5_DMS_SideView/1
  IMAP_Module/323(IMAPve_d_MP5_DMS_EyeFatigue) -> IMAPve_d_MP5_DMS_EyeFatigue/1
  IMAP_Module/324(IMAPve_d_MP5_DMS_LongtimeDrive) -> IMAPve_d_MP5_DMS_LongtimeDrive/1
  IMAP_Module/295(IMAPve_d_ESC_TCS_ErrorStatus) -> IMAPve_d_ESC_TCS_ErrorStatus/1
  IMAP_Module/294(IMAPve_d_ESC_FRW_Direction) -> IMAPve_d_ESC_FRW_Direction/1
  IMAP_Module/304(IMAPve_d_ACU_RearLeft_Belt) -> IMAPve_d_ACU_RearLeft_Belt/1
  IMAP_Module/322(IMAPve_d_MP5_DMS_Sensity) -> IMAPve_d_MP5_DMS_Sensity/1
  IMAP_Module/321(IMAPve_d_MP5_DMS_DelUserNum) -> IMAPve_d_MP5_DMS_DelUserNum/1
  IMAP_Module/309(IMAPve_d_BCM_LeftTurn_Switch) -> IMAPve_d_BCM_LeftTurn_Switch/1
  IMAP_Module/308(IMAPve_d_TCU_TCU_Available) -> IMAPve_d_TCU_TCU_Available/1
  IMAP_Module/296(IMAPve_d_ESC_RLW_Direction) -> IMAPve_d_ESC_RLW_Direction/1
  IMAP_Module/293(IMAPve_d_ESC_FLW_Direction) -> IMAPve_d_ESC_FLW_Direction/1
  IMAP_Module/305(IMAPve_d_ACU_RearMiddle_Belt) -> IMAPve_d_ACU_RearMiddle_Belt/1
  IMAP_Module/313(IMAPve_d_MP5_Work_State) -> IMAPve_d_MP5_Work_State/1
  IMAP_Module/319(IMAPve_d_MP5_DMS_MessageType) -> IMAPve_d_MP5_DMS_MessageType/1
  IMAP_Module/320(IMAPve_d_MP5_DMS_SystemEnable) -> IMAPve_d_MP5_DMS_SystemEnable/1
  IMAP_Module/328(IMAPve_d_MP5_DMS_DrinkWater) -> IMAPve_d_MP5_DMS_DrinkWater/1
  IMAP_Module/312(IMAPve_d_BCM_IHBC_Enabled) -> IMAPve_d_BCM_IHBC_Enabled/1
  IMAP_Module/298(IMAPve_d_ESC_EPB_ErrorStatus) -> IMAPve_d_ESC_EPB_ErrorStatus/1
  IMAP_Module/310(IMAPve_d_BCM_RightTurn_Switch) -> IMAPve_d_BCM_RightTurn_Switch/1
  IMAP_Module/318(IMAPve_d_MP5_AutoPilot_Switch) -> IMAPve_d_MP5_AutoPilot_Switch/1
  IMAP_Module/326(IMAPve_d_MP5_DMS_UsingPhone) -> IMAPve_d_MP5_DMS_UsingPhone/1
  IMAP_Module/301(IMAPve_d_EPS_Driver_Override) -> IMAPve_d_EPS_Driver_Override/1
  IMAP_Module/329(IMAPve_d_MP5_DMS_UserAccount) -> IMAPve_d_MP5_DMS_UserAccount/1
  IMAP_Module/311(IMAPve_d_BCM_FrontWiper_Switch) -> IMAPve_d_BCM_FrontWiper_Switch/1
  IMAP_Module/302(IMAPve_d_EPS_Driver_Active_ESA) -> IMAPve_d_EPS_Driver_Active_ESA/1
  IMAP_Module/303(IMAPve_d_EPS_ESA_State) -> IMAPve_d_EPS_ESA_State/1
  IMAP_Module/317(IMAPve_d_MP5_FLK_Activation) -> IMAPve_d_MP5_FLK_Activation/1
  IMAP_Module/306(IMAPve_d_ACU_RearRight_Belt) -> IMAPve_d_ACU_RearRight_Belt/1
  SWINve_y_Mp5_ISAMode/1 -> IMAP_Module/233(SWINve_y_Mp5_ISAMode)
  SWINve_y_Mp5_LDWWarningMode/1 -> IMAP_Module/234(SWINve_y_Mp5_LDWWarningMode)
  SWINve_y_MP5_ADASSpeedLimit/1 -> IMAP_Module/235(SWINve_y_MP5_ADASSpeedLimit)
  SWINve_y_MP5_TLCModeSelection/1 -> IMAP_Module/236(SWINve_y_MP5_TLCModeSelection)
  SWINve_y_MP5_ESASwitch/1 -> IMAP_Module/237(SWINve_y_MP5_ESASwitch)
  SWINve_y_PEPS_RKECommand/1 -> IMAP_Module/239(SWINve_y_PEPS_RKECommand)
  SWINve_y_MP5_BSD_LCW_Activation/1 -> IMAP_Module/240(SWINve_y_MP5_BSD_LCW_Activation)
  SWINve_y_MP5_FCTAActivation/1 -> IMAP_Module/241(SWINve_y_MP5_FCTAActivation)
  SWINve_y_MP5_RCTAActivation/1 -> IMAP_Module/242(SWINve_y_MP5_RCTAActivation)
  SWINve_y_MP5_DOWActivation/1 -> IMAP_Module/243(SWINve_y_MP5_DOWActivation)
  SWINve_y_MP5_JA_Modes/1 -> IMAP_Module/244(SWINve_y_MP5_JA_Modes)
  SWINve_y_ESC_BLRequest/1 -> IMAP_Module/246(SWINve_y_ESC_BLRequest)
  SWINve_y_PEPS_DoorLockReq/1 -> IMAP_Module/247(SWINve_y_PEPS_DoorLockReq)
  SWINve_y_BCM_DoorLockSt/1 -> IMAP_Module/248(SWINve_y_BCM_DoorLockSt)
  SWINve_y_BCM_LowBeamStatus/1 -> IMAP_Module/249(SWINve_y_BCM_LowBeamStatus)
  SWINve_g_BCM_BattVolt/1 -> IMAP_Module/250(SWINve_g_BCM_BattVolt)
  SWINve_d_TBOX_LocalTimeYear/1 -> IMAP_Module/251(SWINve_d_TBOX_LocalTimeYear)
  SWINve_y_TBOX_LocalTimeMonth/1 -> IMAP_Module/252(SWINve_y_TBOX_LocalTimeMonth)
  SWINve_y_TBOX_LocalTimeDate/1 -> IMAP_Module/253(SWINve_y_TBOX_LocalTimeDate)
  SWINve_y_TBOX_LocalTimeHour/1 -> IMAP_Module/254(SWINve_y_TBOX_LocalTimeHour)
  SWINve_y_TBOX_LocalTimeMinute/1 -> IMAP_Module/255(SWINve_y_TBOX_LocalTimeMinute)
  SWINve_y_TBOX_LocalTimeSecond/1 -> IMAP_Module/256(SWINve_y_TBOX_LocalTimeSecond)
  SWINve_y_TBOX_LocalTimeValid/1 -> IMAP_Module/257(SWINve_y_TBOX_LocalTimeValid)
  SWINve_g_AC_AmbTemp/1 -> IMAP_Module/258(SWINve_g_AC_AmbTemp)
  SWINve_y_EPS_SteeringTorqueSensorSt/1 -> IMAP_Module/259(SWINve_y_EPS_SteeringTorqueSensorSt)
  SWINve_g_EPS_LKACurrentOverlay/1 -> IMAP_Module/260(SWINve_g_EPS_LKACurrentOverlay)
  SWINve_y_ESC_AVHStatus/1 -> IMAP_Module/285(SWINve_y_ESC_AVHStatus)
  SWINve_y_ESC_EBDAlarmSig/1 -> IMAP_Module/284(SWINve_y_ESC_EBDAlarmSig)
  SWINve_y_ESC_EPBSwitchStaticsValidity/1 -> IMAP_Module/283(SWINve_y_ESC_EPBSwitchStaticsValidity)
  SWINve_y_ESC_EPBSwitchStatics/1 -> IMAP_Module/282(SWINve_y_ESC_EPBSwitchStatics)
  SWINve_y_ESC_EPBWarningIndicationReq/1 -> IMAP_Module/281(SWINve_y_ESC_EPBWarningIndicationReq)
  SWINve_y_ESC_EPBDisplayMessageReq/1 -> IMAP_Module/280(SWINve_y_ESC_EPBDisplayMessageReq)
  SWINve_y_ESC_ACCActive/1 -> IMAP_Module/279(SWINve_y_ESC_ACCActive)
  SWINve_y_ESC_ACCAvailable/1 -> IMAP_Module/278(SWINve_y_ESC_ACCAvailable)
  SWINve_y_ESC_AEBActive/1 -> IMAP_Module/277(SWINve_y_ESC_AEBActive)
  SWINve_y_ESC_AEBAvailable/1 -> IMAP_Module/276(SWINve_y_ESC_AEBAvailable)
  SWINve_y_ESC_RRWHeelSpdFaultSignal/1 -> IMAP_Module/275(SWINve_y_ESC_RRWHeelSpdFaultSignal)
  SWINve_y_ESC_RLWHeelSpdFaultSignal/1 -> IMAP_Module/274(SWINve_y_ESC_RLWHeelSpdFaultSignal)
  SWINve_y_ESC_FRWHeelSpdFaultSignal/1 -> IMAP_Module/273(SWINve_y_ESC_FRWHeelSpdFaultSignal)
  SWINve_y_ESC_FLWHeelSpdFaultSignal/1 -> IMAP_Module/272(SWINve_y_ESC_FLWHeelSpdFaultSignal)
  SWINve_y_ESC_ABSAlarmSig/1 -> IMAP_Module/271(SWINve_y_ESC_ABSAlarmSig)
  SWINve_y_ESC_ABSValidity/1 -> IMAP_Module/270(SWINve_y_ESC_ABSValidity)
  SWINve_y_ESC_LongitudinalAccelerationValidity/1 -> IMAP_Module/269(SWINve_y_ESC_LongitudinalAccelerationValidity)
  SWINve_y_ESC_YawrateValidity/1 -> IMAP_Module/268(SWINve_y_ESC_YawrateValidity)
  SWINve_y_ESC_LateralAccelarationValidity/1 -> IMAP_Module/267(SWINve_y_ESC_LateralAccelarationValidity)
  SWINve_y_TCU_ShiftLeverPosValidFlag/1 -> IMAP_Module/266(SWINve_y_TCU_ShiftLeverPosValidFlag)
  SWINve_y_TCU_PRNDLStatus/1 -> IMAP_Module/265(SWINve_y_TCU_PRNDLStatus)
  SWINve_y_EMS_AccPedalFaultBit/1 -> IMAP_Module/264(SWINve_y_EMS_AccPedalFaultBit)
  SWINve_g_EMS_EngActualIndTorque/1 -> IMAP_Module/263(SWINve_g_EMS_EngActualIndTorque)
  SWINve_g_EPS_ElectPowerConsumption/1 -> IMAP_Module/262(SWINve_g_EPS_ElectPowerConsumption)
  SWINve_y_EPS_WarningLampSt/1 -> IMAP_Module/261(SWINve_y_EPS_WarningLampSt)
  SWINve_y_BCM_LeftlightSt/1 -> IMAP_Module/286(SWINve_y_BCM_LeftlightSt)
  SWINve_y_BCM_RightlightSt/1 -> IMAP_Module/287(SWINve_y_BCM_RightlightSt)
  SWINve_y_BCM_TrunkSt/1 -> IMAP_Module/288(SWINve_y_BCM_TrunkSt)
  SWINve_y_BCM_LFDoorSwitchSt/1 -> IMAP_Module/289(SWINve_y_BCM_LFDoorSwitchSt)
  SWINve_y_BCM_RFDoorSwitchSt/1 -> IMAP_Module/290(SWINve_y_BCM_RFDoorSwitchSt)
  SWINve_y_BCM_RRDoorSwitchSt/1 -> IMAP_Module/291(SWINve_y_BCM_RRDoorSwitchSt)
  SWINve_y_BCM_LRDoorSwitchSt/1 -> IMAP_Module/292(SWINve_y_BCM_LRDoorSwitchSt)
  IMAP_Module/331(IMAPva_d_ORI_Obj_TimeStamp) -> IMAPva_d_ORI_Obj_TimeStamp/1
  IMAP_Module/332(IMAPve_d_ORI_FS_OutOfCalib) -> IMAPve_d_ORI_FS_OutOfCalib/1
  IMAP_Module/333(IMAPve_d_ORI_FS_Rain) -> IMAPve_d_ORI_FS_Rain/1
  IMAP_Module/334(IMAPve_d_ORI_FS_Fog) -> IMAPve_d_ORI_FS_Fog/1
  IMAP_Module/335(IMAPve_d_ORI_FS_Splashes0) -> IMAPve_d_ORI_FS_Splashes0/1
  IMAP_Module/336(IMAPve_d_ORI_FS_SunRay0) -> IMAPve_d_ORI_FS_SunRay0/1
  IMAP_Module/337(IMAPve_d_ORI_FS_LowSun0) -> IMAPve_d_ORI_FS_LowSun0/1
  IMAP_Module/338(IMAPve_d_ORI_FS_BlurImage0) -> IMAPve_d_ORI_FS_BlurImage0/1
  IMAP_Module/339(IMAPve_d_ORI_FS_PartialBlockage0) -> IMAPve_d_ORI_FS_PartialBlockage0/1
  IMAP_Module/340(IMAPve_d_ORI_FS_FullBlockage0) -> IMAPve_d_ORI_FS_FullBlockage0/1
  IMAP_Module/341(IMAPve_d_ORI_FS_FrozenWindshield0) -> IMAPve_d_ORI_FS_FrozenWindshield0/1
  IMAP_Module/342(IMAPve_d_ORI_FS_OutOfFocus0) -> IMAPve_d_ORI_FS_OutOfFocus0/1
  IMAP_Module/343(IMAPva_g_ORI_Obj_AbsAx) -> IMAPva_g_ORI_Obj_AbsAx/1
  IMAP_Module/344(IMAPva_g_ORI_Obj_AbsAy) -> IMAPva_g_ORI_Obj_AbsAy/1
  IMAP_Module/345(IMAPva_g_ORI_Obj_RelVely) -> IMAPva_g_ORI_Obj_RelVely/1
  IMAP_Module/346(IMAPva_g_ORI_Obj_LateralDis) -> IMAPva_g_ORI_Obj_LateralDis/1
  IMAP_Module/347(IMAPva_g_ORI_Obj_AbsAxStdDev) -> IMAPva_g_ORI_Obj_AbsAxStdDev/1
  IMAP_Module/348(IMAPva_g_ORI_Obj_AbsAyStdDev) -> IMAPva_g_ORI_Obj_AbsAyStdDev/1
  IMAP_Module/349(IMAPva_g_ORI_Obj_RelVelStdDev) -> IMAPva_g_ORI_Obj_RelVelStdDev/1
  IMAP_Module/350(IMAPva_g_ORI_Obj_RelVelyStdDev) -> IMAPva_g_ORI_Obj_RelVelyStdDev/1
  IMAP_Module/351(IMAPva_g_ORI_Obj_LongDisStdDev) -> IMAPva_g_ORI_Obj_LongDisStdDev/1
  IMAP_Module/352(IMAPva_g_ORI_Obj_LateralDisStdDev) -> IMAPva_g_ORI_Obj_LateralDisStdDev/1
  IMAP_Module/353(IMAPva_d_ORI_Obj_RelVelValid) -> IMAPva_d_ORI_Obj_RelVelValid/1
  IMAP_Module/354(IMAPva_d_ORI_Obj_RelVelyValid) -> IMAPva_d_ORI_Obj_RelVelyValid/1
  IMAP_Module/355(IMAPva_d_ORI_Obj_RelVelStdDevValid) -> IMAPva_d_ORI_Obj_RelVelStdDevValid/1
  IMAP_Module/356(IMAPva_d_ORI_Obj_RelVelyStdDevValid) -> IMAPva_d_ORI_Obj_RelVelyStdDevValid/1
  IMAP_Module/357(IMAPva_g_ORI_Obj_ExistProb) -> IMAPva_g_ORI_Obj_ExistProb/1
  IMAP_Module/359(IMAPva_g_ORI_Obj_Height) -> IMAPva_g_ORI_Obj_Height/1
  IMAP_Module/360(IMAPva_g_ORI_Obj_LengthStdDev) -> IMAPva_g_ORI_Obj_LengthStdDev/1
  IMAP_Module/361(IMAPva_g_ORI_Obj_WidthStdDev) -> IMAPva_g_ORI_Obj_WidthStdDev/1
  IMAP_Module/362(IMAPva_g_ORI_Obj_HeightStdDev) -> IMAPva_g_ORI_Obj_HeightStdDev/1
  IMAP_Module/363(IMAPva_g_ORI_Obj_3DAngle) -> IMAPva_g_ORI_Obj_3DAngle/1
  IMAP_Module/364(IMAPva_g_ORI_Obj_LAngleStdDev) -> IMAPva_g_ORI_Obj_LAngleStdDev/1
  IMAP_Module/365(IMAPva_g_ORI_Obj_RAngleStdDev) -> IMAPva_g_ORI_Obj_RAngleStdDev/1
  IMAP_Module/366(IMAPva_g_ORI_Obj_3DAngleStdDev) -> IMAPva_g_ORI_Obj_3DAngleStdDev/1
  IMAP_Module/367(IMAPva_g_ORI_Obj_AngleRate) -> IMAPva_g_ORI_Obj_AngleRate/1
  IMAP_Module/368(IMAPva_g_ORI_Obj_AngleRateStdDev) -> IMAPva_g_ORI_Obj_AngleRateStdDev/1
  IMAP_Module/369(IMAPva_g_ORI_Obj_PhiBottom) -> IMAPva_g_ORI_Obj_PhiBottom/1
  IMAP_Module/370(IMAPva_g_ORI_Obj_PhiBottomStdDev) -> IMAPva_g_ORI_Obj_PhiBottomStdDev/1
  IMAP_Module/371(IMAPva_d_ORI_Obj_Measured) -> IMAPva_d_ORI_Obj_Measured/1
  IMAP_Module/372(IMAPva_g_ORI_Obj_Heading) -> IMAPva_g_ORI_Obj_Heading/1
  IMAP_Module/373(IMAPva_g_ORI_Obj_HeadingStdDev) -> IMAPva_g_ORI_Obj_HeadingStdDev/1
  IMAP_Module/374(IMAPva_d_ORI_Obj_HeadOrientation) -> IMAPva_d_ORI_Obj_HeadOrientation/1
  IMAP_Module/376(IMAPva_g_ORI_Obj_TTIPCStdDev) -> IMAPva_g_ORI_Obj_TTIPCStdDev/1
  IMAP_Module/375(IMAPva_g_ORI_Obj_TTIPC) -> IMAPva_g_ORI_Obj_TTIPC/1
  IMAP_Module/377(IMAPva_d_ORI_Obj_DirectionIndicator) -> IMAPva_d_ORI_Obj_DirectionIndicator/1
  IMAP_Module/378(IMAPva_d_ORI_Obj_BrakeLight) -> IMAPva_d_ORI_Obj_BrakeLight/1
  IMAP_Module/379(IMAPve_d_ORI_L0_ID) -> IMAPve_d_ORI_L0_ID/1
  IMAP_Module/380(IMAPve_g_ORI_L0_ExistProb) -> IMAPve_g_ORI_L0_ExistProb/1
  IMAP_Module/381(IMAPve_g_ORI_L0_DxStart) -> IMAPve_g_ORI_L0_DxStart/1
  IMAP_Module/382(IMAPve_d_ORI_L0_ColorClass) -> IMAPve_d_ORI_L0_ColorClass/1
  IMAP_Module/383(IMAPve_d_ORI_L0_MeasureType) -> IMAPve_d_ORI_L0_MeasureType/1
  IMAP_Module/384(IMAPve_g_ORI_L0_TypeConf) -> IMAPve_g_ORI_L0_TypeConf/1
  IMAP_Module/385(IMAPve_d_ORI_R0_ID) -> IMAPve_d_ORI_R0_ID/1
  IMAP_Module/386(IMAPve_g_ORI_R0_ExistProb) -> IMAPve_g_ORI_R0_ExistProb/1
  IMAP_Module/387(IMAPve_g_ORI_R0_Dxstart) -> IMAPve_g_ORI_R0_Dxstart/1
  IMAP_Module/388(IMAPve_d_ORI_R0_ColorClass) -> IMAPve_d_ORI_R0_ColorClass/1
  IMAP_Module/389(IMAPve_d_ORI_R0_MeasureType) -> IMAPve_d_ORI_R0_MeasureType/1
  IMAP_Module/390(IMAPve_g_ORI_R0_TypeConf) -> IMAPve_g_ORI_R0_TypeConf/1
  IMAP_Module/391(IMAPve_d_ORI_L1_ID) -> IMAPve_d_ORI_L1_ID/1
  IMAP_Module/392(IMAPve_g_ORI_L1_ExistProb) -> IMAPve_g_ORI_L1_ExistProb/1
  IMAP_Module/393(IMAPve_g_ORI_L1_Dxstart) -> IMAPve_g_ORI_L1_Dxstart/1
  IMAP_Module/394(IMAPve_d_ORI_L1_ColorClass) -> IMAPve_d_ORI_L1_ColorClass/1
  IMAP_Module/395(IMAPve_d_ORI_L1_MeasureType) -> IMAPve_d_ORI_L1_MeasureType/1
  IMAP_Module/396(IMAPve_g_ORI_L1_TypeConf) -> IMAPve_g_ORI_L1_TypeConf/1
  IMAP_Module/397(IMAPve_d_ORI_R1_ID) -> IMAPve_d_ORI_R1_ID/1
  IMAP_Module/398(IMAPve_g_ORI_R1_ExistProb) -> IMAPve_g_ORI_R1_ExistProb/1
  IMAP_Module/399(IMAPve_g_ORI_R1_Dxstart) -> IMAPve_g_ORI_R1_Dxstart/1
  IMAP_Module/400(IMAPve_d_ORI_R1_ColorClass) -> IMAPve_d_ORI_R1_ColorClass/1
  IMAP_Module/401(IMAPve_d_ORI_R1_MeasureType) -> IMAPve_d_ORI_R1_MeasureType/1
  IMAP_Module/402(IMAPve_g_ORI_R1_TypeConf) -> IMAPve_g_ORI_R1_TypeConf/1
  IMAP_Module/403(IMAPve_d_ORI_RoadedgeL0_ID) -> IMAPve_d_ORI_RoadedgeL0_ID/1
  IMAP_Module/404(IMAPve_g_ORI_RoadedgeL0_ExistProb) -> IMAPve_g_ORI_RoadedgeL0_ExistProb/1
  IMAP_Module/405(IMAPve_g_ORI_RoadedgeL0_DxStart) -> IMAPve_g_ORI_RoadedgeL0_DxStart/1
  IMAP_Module/406(IMAPve_g_ORI_RoadedgeL0_DxEnd) -> IMAPve_g_ORI_RoadedgeL0_DxEnd/1
  IMAP_Module/407(IMAPve_g_ORI_RoadedgeL0_C1) -> IMAPve_g_ORI_RoadedgeL0_C1/1
  IMAP_Module/408(IMAPve_g_ORI_RoadedgeL0_C0) -> IMAPve_g_ORI_RoadedgeL0_C0/1
  IMAP_Module/409(IMAPve_g_ORI_RoadedgeL0_C3) -> IMAPve_g_ORI_RoadedgeL0_C3/1
  IMAP_Module/410(IMAPve_g_ORI_RoadedgeL0_C2) -> IMAPve_g_ORI_RoadedgeL0_C2/1
  IMAP_Module/411(IMAPve_d_ORI_RoadedgeL0_MeasureType) -> IMAPve_d_ORI_RoadedgeL0_MeasureType/1
  IMAP_Module/412(IMAPve_d_ORI_RoadedgeL0_Type) -> IMAPve_d_ORI_RoadedgeL0_Type/1
  IMAP_Module/413(IMAPve_d_ORI_RoadedgeR0_ID) -> IMAPve_d_ORI_RoadedgeR0_ID/1
  IMAP_Module/414(IMAPve_g_ORI_RoadedgeR0_ExistProb) -> IMAPve_g_ORI_RoadedgeR0_ExistProb/1
  IMAP_Module/415(IMAPve_g_ORI_RoadedgeR0_DxStart) -> IMAPve_g_ORI_RoadedgeR0_DxStart/1
  IMAP_Module/416(IMAPve_g_ORI_RoadedgeR0_DxEnd) -> IMAPve_g_ORI_RoadedgeR0_DxEnd/1
  IMAP_Module/417(IMAPve_g_ORI_RoadedgeR0_C1) -> IMAPve_g_ORI_RoadedgeR0_C1/1
  IMAP_Module/418(IMAPve_g_ORI_RoadedgeR0_C0) -> IMAPve_g_ORI_RoadedgeR0_C0/1
  IMAP_Module/419(IMAPve_g_ORI_RoadedgeR0_C3) -> IMAPve_g_ORI_RoadedgeR0_C3/1
  IMAP_Module/420(IMAPve_g_ORI_RoadedgeR0_C2) -> IMAPve_g_ORI_RoadedgeR0_C2/1
  IMAP_Module/421(IMAPve_d_ORI_RoadedgeR0_MeasureType) -> IMAPve_d_ORI_RoadedgeR0_MeasureType/1
  IMAP_Module/422(IMAPve_d_ORI_RoadedgeR0_Type) -> IMAPve_d_ORI_RoadedgeR0_Type/1
  IMAP_Module/358(IMAPva_g_ORI_Obj_ClassProb) -> IMAPva_g_ORI_Obj_ClassProb/1
  SWINve_g_ESC_BrakeWheelCylinderPressure/1 -> IMAP_Module/293(SWINve_g_ESC_BrakeWheelCylinderPressure)
  IMAP_Module/330(IMAPve_g_ESC_BrkWhlCylinder_Pressure) -> IMAPve_g_ESC_BrkWhlCylinder_Pressure/1
  IMAP_Module/423(IMAPve_d_APA_AutoPark_WorkSt) -> IMAPve_d_APA_AutoPark_WorkSt/1
  FAPAve_Cnt_AdvancedParkingAssist/1 -> IMAP_Module/294(FAPAve_Cnt_AdvancedParkingAssist)
  IMAP_Module/424(IMAPve_g_ob020H_100) -> IMAPve_g_ob020H_100/1
  IMAP_Module/425(IMAPve_g_ob020L_100) -> IMAPve_g_ob020L_100/1
  SWINve_y_MP5_JA_Alert_Switch/1 -> IMAP_Module/245(SWINve_y_MP5_JA_Alert_Switch)
  SWINve_y_Mp5_ELKSwitch/1 -> IMAP_Module/238(SWINve_y_Mp5_ELKSwitch)
  SDFAve_y_ISASignType/1 -> IMAP_Module/189(SDFAve_y_ISASignType)
  SDFAve_y_ISAStatus/1 -> IMAP_Module/190(SDFAve_y_ISAStatus)
  SDFAve_y_ISAPopupMessage/1 -> IMAP_Module/188(SDFAve_y_ISAPopupMessage)
  IMAP_Module/285(IMAPve_d_ISA_Popup_Message) -> IMAPve_d_ISA_Popup_Message/1
  IMAP_Module/286(IMAPve_d_ISA_Sign_Type) -> IMAPve_d_ISA_Sign_Type/1
  IMAP_Module/287(IMAPve_d_ISA_Status) -> IMAPve_d_ISA_Status/1
  SDFAve_y_Radar_State/1 -> IMAP_Module/193(SDFAve_y_Radar_State)
  SDFAve_y_OperatingStatus/1 -> IMAP_Module/194(SDFAve_y_OperatingStatus)
  IMAP_Module/290(IMAPve_d_Camera_State) -> IMAPve_d_Camera_State/1
  SDFAve_d_fusion_status/1 -> IMAP_Module/96(SDFAve_d_fusion_status)
  IMAP_Module/193(IMAPve_d_Fusion_Status) -> IMAPve_d_Fusion_Status/1
  SDFAve_y_Radar_FaultBitSetting_Signal/1 -> IMAP_Module/195(SDFAve_y_Radar_FaultBitSetting_Signal)
  IMAP_Module/291(IMAPve_d_Radar_FaultBitSetting_Signal) -> IMAPve_d_Radar_FaultBitSetting_Signal/1
  SDFAva_g_ORI_Obj_LongDis/1 -> IMAP_Module/303(SDFAva_d_ORI_Obj_Class)
  SDFAve_g_ORI_L1_C2/1 -> IMAP_Module/312(SDFAve_g_ORI_L1_C2)
  SDFAve_g_ORI_L0_C1/1 -> IMAP_Module/307(SDFAve_g_ORI_L0_C1)
  SDFAve_g_ORI_L0_C3/1 -> IMAP_Module/305(SDFAve_g_ORI_L0_C3)
  SDFAva_d_ORI_Obj_Class/1 -> IMAP_Module/297(SDFAva_g_ORI_Obj_AbsAx)
  SDFAva_d_ORI_Obj_ID/1 -> IMAP_Module/298(SDFAva_g_ORI_Obj_AbsAy)
  SDFAve_g_ORI_R1_C2/1 -> IMAP_Module/324(SDFAve_g_ORI_R1_C2)
  SDFAve_g_ORI_R1_VR/1 -> IMAP_Module/328(SDFAve_g_ORI_R1_VR)
  SDFAva_g_ORI_Obj_AbsAy/1 -> IMAP_Module/300(SDFAva_g_ORI_Obj_RelVely)
  SDFAve_g_ORI_R1_C1/1 -> IMAP_Module/325(SDFAve_g_ORI_R1_C1)
  SDFAve_g_ORI_L1_VR/1 -> IMAP_Module/316(SDFAve_g_ORI_L1_VR)
  SDFAve_g_ORI_L1_C0/1 -> IMAP_Module/314(SDFAve_g_ORI_L1_C0)
  SDFAve_g_ORI_L1_C1/1 -> IMAP_Module/313(SDFAve_g_ORI_L1_C1)
  SDFAva_g_ORI_Obj_LateralDis/1 -> IMAP_Module/304(SDFAva_d_ORI_Obj_ID)
  SDFAve_g_ORI_L1_C3/1 -> IMAP_Module/311(SDFAve_g_ORI_L1_C3)
  SDFAve_g_ORI_R1_C0/1 -> IMAP_Module/326(SDFAve_g_ORI_R1_C0)
  SDFAve_g_ORI_R0_C0/1 -> IMAP_Module/320(SDFAve_g_ORI_R0_C0)
  SDFAva_g_ORI_Obj_RelVel/1 -> IMAP_Module/301(SDFAva_g_ORI_Obj_LongDis)
  SDFAve_g_ORI_R0_C2/1 -> IMAP_Module/318(SDFAve_g_ORI_R0_C2)
  SDFAve_g_ORI_L0_C0/1 -> IMAP_Module/308(SDFAve_g_ORI_L0_C0)
  SDFAve_g_ORI_L0_VR/1 -> IMAP_Module/310(SDFAve_g_ORI_L0_VR)
  SDFAve_d_ORI_R0_LT/1 -> IMAP_Module/321(SDFAve_d_ORI_R0_LT)
  SDFAve_g_ORI_R0_VR/1 -> IMAP_Module/322(SDFAve_g_ORI_R0_VR)
  SDFAve_d_ORI_R1_LT/1 -> IMAP_Module/327(SDFAve_d_ORI_R1_LT)
  SDFAve_d_ORI_CIPV_ID/1 -> IMAP_Module/295(SDFAve_d_ORI_CIPV_ID)
  SDFAve_d_ORI_L1_Type/1 -> IMAP_Module/315(SDFAve_d_ORI_L1_Type)
  SDFAve_g_ORI_R0_C3/1 -> IMAP_Module/317(SDFAve_g_ORI_R0_C3)
  SDFAva_g_ORI_Obj_RelVely/1 -> IMAP_Module/302(SDFAva_g_ORI_Obj_LateralDis)
  SDFAve_g_ORI_R1_C3/1 -> IMAP_Module/323(SDFAve_g_ORI_R1_C3)
  SDFAve_g_ORI_L0_C2/1 -> IMAP_Module/306(SDFAve_g_ORI_L0_C2)
  SDFAva_g_ORI_Obj_AbsAx/1 -> IMAP_Module/299(SDFAva_g_ORI_Obj_RelVel)
  SDFAve_d_ORI_L0_Type/1 -> IMAP_Module/309(SDFAve_d_ORI_L0_Type)
  SDFAve_d_ORI_Obj_Num/1 -> IMAP_Module/296(SDFAve_d_ORI_Obj_Num)
  SDFAve_g_ORI_R0_C1/1 -> IMAP_Module/319(SDFAve_g_ORI_R0_C1)
